simulink model "mcb_microchip_pmsm_foc_sensorless_SAME54_pot"  (R2023b)
settings: Solver=FixedStepDiscrete  StartTime=0.0  StopTime=5  FixedStep=Ts  RelTol=1e-3  EnableMultiTasking=on
InitFcn:
  | mcb_microchip_pmsm_foc_sensorless_SAME54_data
values from neighbouring files (symbols this model uses):
  PI_params = mcb.internal.SetControllerParameters(pmsm,inverter,PU_System,T_pwm,2*Ts,Ts_speed)    [mcb_microchip_pmsm_foc_sensorless_SAME54_data.m]
  PU_System = mcb_SetPUSystem(pmsm,inverter)    [mcb_microchip_pmsm_foc_sensorless_SAME54_data.m]
  PWM_frequency = 12e3    (= 12000)    [mcb_microchip_pmsm_foc_sensorless_SAME54_data.m]
  Ts = T_pwm    (= 8.33333333333e-05)    [mcb_microchip_pmsm_foc_sensorless_SAME54_data.m]
  Ts_motor = T_pwm    (= 8.33333333333e-05)    [mcb_microchip_pmsm_foc_sensorless_SAME54_data.m]
  Ts_simulink = T_pwm    (= 8.33333333333e-05)    [mcb_microchip_pmsm_foc_sensorless_SAME54_data.m]
  Ts_speed = 10*Ts    (= 0.000833333333333)    [mcb_microchip_pmsm_foc_sensorless_SAME54_data.m]
  Vd_Ref_openLoop_PU = 0.15    [mcb_microchip_pmsm_foc_sensorless_SAME54_data.m]
undefined symbols (not defined in the file or in its folder): AIN0, AIN6, DiscIntNeverNeededParam, inverter, PA02, PA03, PA06, PA08, PA09, PA10, PA11, PA12, PA13, PA16, PA17, PA18, pad0, pad1, pad2, pad3, PB08, Pin, pmsm, SAME54P20A, Timer, TQFP128, VREFA, wo0, wo1, wo2, wo4, wo5, wo6
libraries: simulink x16, MCHP_Blockset x15, mcbcontrolslib x10, slpidlib x3, mcbpositiondecoderlib x2, mcbsensorlessestimatorlib x1, mcbplantlib x1, autolibpmsmexterior x1
(part 2 of 4)

== system mcb_microchip_pmsm_foc_sensorless_SAME54_pot/Configurations ==
  note: PIM: https://www.microchip.com/Developmenttools/ProductDetails/MA320203
  note: MCLV-2				SAME70-PIM
      | --------------------------------------------------
      | DBG_LED1			PC23
      | DBG_LED2			PA24
      |
      | Rx					PA09_URXD0
      | Tx					PA10_UTXD0
      |
      | HALLA				PA00 - PD13
      | HALLB				PA01 - PD10
      | HALLC				PA16 - PD11
      |
      | PWM1				PD24 (L) - PA11 (H)
      | PWM2				PD25 (L) - PA12 (H)
      | PWM3				PD26 (L) - PA13 (H)
      |
      | FAULT				PD09_FAULT_PWM
      |
      | POT				PB00 (not ok on early PIMs)
      | PUSH S2			PC03
      | PUSH S3			PC01
      |
      | PIM_V_M1			PD30
      | PIM_V_M2			PA17
      | PIM_V_M3			PA21 - PA19
  Compiler Options : MCHP_Blockset/System Configuration/Compiler Options  Priority=1  LATEST_CMPLR=on  COMP_LIST=Dynamic Options  COMP_LIST_TXT=xc32 - v4.30  DFP_LIST=Dynamic Options  DFP_LIST_TXT=v 3.8.234  CMSIS_DSP=Dynamic Options  CMSIS_DSP_TXT=Not used  USE_64BIT_DOUBLE=off  MCHP_MULTITHREAD_COMPILATION=on  UseCustom_LinkerScript=off  MCHP_MASTERLINK=mcb_microchip_pmsm_foc_sensorless_SAME54_pot1/Configurations/Microchip Master  OPTIMIZATION_LEVEL=3  MPLAB_LINKLIB=default  MPLAB_LINKLIB1=default  CodeReplacement=Dynamic Options  CodeReplacement_TXT=None  OPTIMIZATION_FLTO=off  OPTIMIZATION_REORDER=off  UNROLL_LOOPS=on  PROCEDURAL_ABSTRACTION=off  MCODE=is less than 32768 (faster)  MCONST=in data memory  MDATA=Use only memory below address 8192 (faster)  MSCALAR=Use only memory below address 8192 (faster)  MLARGEARRAY=off  MAGGREGATE=off  HEAP_SIZE=0  OMF=elf  DEBUG_INFO=on  ProduceHexOutput=off  AssemblyListing=off  SaveTemps=off  NO_EDS_WARN=on  PRINT_STATISTICS=off
      settings: SourceProductName=MPLAB Device Blocks for Simulink
  Microchip Master : MCHP_Blockset/System Configuration/Microchip Master  Priority=1  PICREF=SAME54P20A - TQFP128  TIMESTEP_REF="Timer  ( 8.3333e-05s )"  BUSYFLAG=Dynamic Options  BUSYFLAG_TXT=None  VDD_range=Dynamic Options  PWRTEN=Not used  BOREN=Disable  BODENV=2.7V  BORV=Not used  FPWRT=64ms  DSBOREN=Enable ZPBOR during Deep Sleep Mode  DSLPBOR=Not used  MCLRE=Enabled  SMCLR=MCLR pin generates a normal system Reset  PMDL1WAY=Allow only one reconfiguration  RSTPRI=Device will obtain reset instruction from Primary flash  TEMP=Not used  SOSCSRC=Not used  SOSCSEL=Not used  IOL1WAY=Allow only one reconfiguration  ALTVREF=Not used  DISUVREG=Not used  DSSWEN=Not used  LPCFG=Not used  RTCBAT=Not used  VBTBOR=Not used  WUTSEL=Not used  POWERSAVE=off  FNOSC=Primary Oscillator with PLL module (XT + PLL; HS + PLL; EC + PLL)  FPR=ECIO w/ PLL 16x  FOSFPR=HS3 w/PLL 16x  FOS=Internal Fast RC  FRANGE=High Range  OSCILLATOR_SELECT=Crystal Oscillator in 8-48MHz on XIN/XOUT 0  OSCILLATOR_SELECT_spd=Crystal Oscillator in 8-48MHz on XIN/XOUT 0  QUARTZ=12e6  QUARTZ_spd=12e6  POSCGAIN=2x gain setting  POSCBOOST=Boost the kick start of the oscillator  SOSCGAIN=2x gain setting  SOSCBOOST=Boost the kick start of the oscillator  ACTIV_PLL=on  ACTIV_PLL_spd=on  MIPS_DESIRED=120e6  MIPS_DESIRED_spd=120e6  CPUDIV=Divide by 1  FPLLMUL=Not used  FPLLIDIV=8x Divider  POSCFREQ=Not used  POSCMD=Primary Oscillator Disabled  POSCMOD=Primary osc disabled  MIPS=120 * 1e6  ACLKCON=Optimized for PWM resolution & ADC conversion speed  ACLKCON_spd=Optimized for PWM resolution & ADC conversion speed  ACLKCON_Info=use FRC with auxilliary PLL, ADC Tad = 16.961(ns), PWM max resolution = 1.06(ns)  FPLLODIV=32x Divider  PLLKEN=Clock switch to PLL source will wait until the PLL lock signal is valid  FCKSM=Both Clock switching and Fail-safe Clock Monitor are disabled  FCKSMEN=Sw Disabled; Mon Disabled  IESO=Start up with FRC; then switch  DSWDTPS=1:2^36  FWDTEN=Disable  FWDTWINSZ=Window size is 25%  FWPSA=1:512  FWPSA0=1:128  FWPSB=1:16  WDT=Disable  WDTPOST=1:32768  WDTPRE=1:128  WDTPS=1:1048576  WINDIS=Watchdog Timer in Non-Window mode  WWDTEN=Non-Window mode  DSWDTEN=Enable DSWDT during Deep Sleep Mode  DSWDTOSC=Select LPRC as DSWDT Reference clock  FWDT_RCLKSEL=WDT Run Mode uses BFRC:256  FWDT_RWDTPS=1:2147483648  FWDT_SWDTMPS=1:2147483648  FWDT_WDTEN=WDT is controlled by software; use WDTCON.ON bit  FWDT_WDTRSTEN=WDT event generates a reset  FWDT_WDTWIN=WDT Window is 25% of WDT period  FWDT_WINEN=Watchdog Timer operates in Window mode  FPBDIV=Not used  FSOSCEN=Disable Secondary Oscillator  LPRCSEL=Not used  OSCIOFCN=Not used  OSCIOFNC=OSC2 is clock output  LVRCFG=Not used  PLL_96MHZ=Not used  PLL96MHZ=Not used  PLLDIV=Not used  WDTCLK=Not used  WDTCMX=Not used  WDTWIN=WDT Window is 25% of WDT period  XTCFG=24-32 MHz crystals  XTBST=Boost the kick-start  APL=Aux Flash Code protect is disabled  APLK=Aux Flash Write Protection or Code Protection is Enabled  AWRP=Auxiliary program memory is not write-protected  BSS=No Protection (other than BWRP)  BWP=Not used  BWRP=Boot Segment may be written  CP=Protection Disabled  EBS=No Boot EEPROM  ESS=No Segment Data EEPROM  GCP=Disable  GSS=No Protection (other than GWRP)  GSS0=Not used  GSSK=General Segment Write Protection or Code Protection is Enabled  GWRP=General Segment may be written  PWP=Not used  RBS=No Boot RAM  RSS=No Secure RAM  SSS=No Secure Segment  SWRP=Secure segment may be written  WPCFG=Not used  WPDIS=Not used  WPEND=Not used  WPFP=Not used  ICESEL=Communicate on PGEC1/PGED1  ICS=Communicate on PGEC1 and PGED1  JTAGEN=Disable  FICD_JTAGEN=Disable  COE=Not used  RES=Not used  DEBUG=Debugger is disabled  BACKBUG=Not used  BKBUG=Not used  ALTI2C=I2C mapped to SDA1/SCL1 pins  ALTI2C1=I2C1 mapped to SDA1/SCL1 pins  ALTI2C2=I2C2 mapped to SDA2/SCL2 pins  ALTI2C3=I2C3 mapped to SDA3/SCL3 pins  FDEVOPT1_ALTI2C1=Primary I2C1 pins are used  FDEVOPT1_ALTI2C2=Primary I2C2 pins are used  FDEVOPT1_SPI2MAPDIS=SPI2 pins are selected by peripheral pin selection feature  ALTQIO=QEA1; QEB1; INDX1 are selected as inputs to QEI1  ALTSS1=SS1A is selected as the I/O pin for SPI1  CMPPOL0=Hysteresis is applied to falling edge  CMPPOL1=Hysteresis is applied to falling edge  FCANIO=Not used  FETHIO=Default Ethernet I/O  FMIIEN=MII Enabled  FSRSSEL=Not used  FUSBIDIO=Controlled by the USB Module  FVBUSONIO=Not used  HPOL=Active High  HYST0=45 mV Hysteresis  HYST1=45 mV Hysteresis  I2C1SEL=Not used  LPOL=Active High  PWMPIN=Control with PORT/TRIS regs  RTCOSC=Not used  UPLLEN=USB PLL Disabled  UPLLIDIV=Not used  ATMOD8=Not used  ALTPMP=Not used  I2C2SEL=Not used  ALTADREF=Not used  ALTCVREF=Not used  PWMLOCK=PWM registers may be written without key sequence  INT_PRIORITY_DMA=0  MCHP_TIMER_RESULT=[1 8748.999999999992724 ]  MCHP_PLLRegisters="[5    243  16387     -1     -1]"  MCHPVAR=MCHP.id.name='SAME54P20A';MCHP.id.N=reshape([54 20 -1],1,3);MCHP.id.L=reshape({ 'SAME','P','A'},1,3);MCHP.id.maskset='';MCHP.id.dos='';MCHP.id.ds='';MCHP.id.archTxt='';MCHP.id.clonedfrom='';MCHP.id.Arch=6;MCHP.id.pinout=reshape({ 'TFBGA120','TQFP128'},1,2);MCHP.Rx=reshape([1 125 3 13 -1 -1 -1 -1 -1 -1 -1 -1 -1 -1 -1 -1 -1 -1 -1 -1 -1 2 126 4 16 -1 -1 -1 -1 -1 -1 -1 -1 -1 -1 -1 -1 -1 -1 -1 -1 -1 9 127 7 -1 -1 -1 -1 -1 -1 -1 -1 -1 -1 -1 -1 -1 -1 -1 -1 -1 -1 10 128 8 -1 -1 -1 -1 -1 -1 -1 -1 -1 -1 -1 -1 -1 -1 -1 -1 -1 -1 21 11 27 -1 -1 -1 -1 -1 -1 -1 -1 -1 -1 -1 -1 -1 -1 -1 -1 -1 -1 22 12 28 -1 -1 -1 -1 -1 -1 -1 -1 -1 -1 -1 -1 -1 -1 -1 -1 -1 -1 23 17 29 -1 -1 -1 -1 -1 -1 -1 -1 -1 -1 -1 -1 -1 -1 -1 -1 -1 -1 24 18 30 -1 -1 -1 -1 -1 -1 -1 -1 -1 -1 -1 -1 -1 -1 -1 -1 -1 -1 33 19 -1 47 -1 -1 -1 -1 -1 -1 -1 -1 -1 -1 -1 -1 -1 -1 -1 -1 -1 34 20 -1 48 -1 -1 -1 -1 -1 -1 -1 -1 -1 -1 -1 -1 -1 -1 -1 -1 -1 35 39 52 49 -1 -1 -1 -1 -1 -1 -1 -1 -1 -1 -1 -1 -1 -1 -1 -1 -1 36 40 55 50 -1 -1 -1 -1 -1 -1 -1 -1 -1 -1 -1 -1 -1 -1 -1 -1 -1 60 41 56 51 -1 -1 -1 -1 -1 -1 -1 -1 -1 -1 -1 -1 -1 -1 -1 -1 -1 61 42 57 -1 -1 -1 -1 -1 -1 -1 -1 -1 -1 -1 -1 -1 -1 -1 -1 -1 -1 62 43 58 -1 -1 -1 -1 -1 -1 -1 -1 -1 -1 -1 -1 -1 -1 -1 -1 -1 -1 63 44 59 -1 -1 -1 -1 -1 -1 -1 -1 -1 -1 -1 -1 -1 -1 -1 -1 -1 -1 66 82 70 -1 -1 -1 -1 -1 -1 -1 -1 -1 -1 -1 -1 -1 -1 -1 -1 -1 -1 67 83 71 -1 -1 -1 -1 -1 -1 -1 -1 -1 -1 -1 -1 -1 -1 -1 -1 -1 -1 68 84 72 -1 -1 -1 -1 -1 -1 -1 -1 -1 -1 -1 -1 -1 -1 -1 -1 -1 -1 69 85 73 -1 -1 -1 -1 -1 -1 -1 -1 -1 -1 -1 -1 -1 -1 -1 -1 -1 -1 88 86 74 80 -1 -1 -1 -1 -1 -1 -1 -1 -1 -1 -1 -1 -1 -1 -1 -1 -1 89 87 75 81 -1 -1 -1 -1 -1 -1 -1 -1 -1 -1 -1 -1 -1 -1 -1 -1 -1 92 98 76 -1 -1 -1 -1 -1 -1 -1 -1 -1 -1 -1 -1 -1 -1 -1 -1 -1 -1 93 99 77 -1 -1 -1 -1 -1 -1 -1 -1 -1 -1 -1 -1 -1 -1 -1 -1 -1 -1 94 100 108 -1 -1 -1 -1 -1 -1 -1 -1 -1 -1 -1 -1 -1 -1 -1 -1 -1 -1 95 101 109 -1 -1 -1 -1 -1 -1 -1 -1 -1 -1 -1 -1 -1 -1 -1 -1 -1 -1 -1 102 110 -1 -1 -1 -1 -1 -1 -1 -1 -1 -1 -1 -1 -1 -1 -1 -1 -1 -1 113 103 111 -1 -1 -1 -1 -1 -1 -1 -1 -1 -1 -1 -1 -1 -1 -1 -1 -1 -1 -1 104 112 -1 -1 -1 -1 -1 -1 -1 -1 -1 -1 -1 -1 -1 -1 -1 -1 -1 -1 -1 105 -1 -1 -1 -1 -1 -1 -1 -1 -1 -1 -1 -1 -1 -1 -1 -1 -1 -1 -1 119 121 123 -1 -1 -1 -1 -1 -1 -1 -1 -1 -1 -1 -1 -1 -1 -1 -1 -1 -1 120 122 124 -1 -1 -1 -1 -1 -1 -1 -1 -1 -1 -1 -1 -1 -1 -1 -1 -1 -1],21,32);MCHP.memory.FLASH.size=1048576;MCHP.memory.SW0.size=16;MCHP.memory.TEMP_LOG.size=512;MCHP.memory.USER_PAGE.size=512;MCHP.memory.CMCC.size=16777216;MCHP.memory.CMCC_DATARAM.size=4096;MCHP.memory.CMCC_TAGRAM.size=1024;MCHP.memory.CMCC_VALIDRAM.size=64;MCHP.memory.QSPI.size=16777216;MCHP.memory.HSRAM.size=262144;MCHP.memory.HSRAM_ETB.size=32768;MCHP.memory.HSRAM_RET1.size=32768;MCHP.memory.HPB0.size=17408;MCHP.memory.HPB1.size=139264;MCHP.memory.HPB2.size=15360;MCHP.memory.HPB3.size=12288;MCHP.memory.SEEPROM.size=131072;MCHP.memory.SDHC0.size=3072;MCHP.memory.SDHC1.size=3072;MCHP.memory.BKUPRAM.size=8192;MCHP.memory.PPB.size=1048576;MCHP.memory.SCS.size=4096;MCHP.memory.PERIPHERALS.size=MCHP_Fun.Hex2num('41C0000000000000');MCHP.module.PM.PID=0;MCHP.module.PM.vector='PM';MCHP.module.MCLK.PID=1;MCHP.module.MCLK.vector='MCLK';MCHP.module.OSCCTRL(1).PID=2;MCHP.module.OSCCTRL(1).vector='OSCCTRL_XOSC0';MCHP.module.OSCCTRL(1).pin.XIN0.txt={ 'PA14'};MCHP.module.OSCCTRL(1).pin.XIN0.Rx_idx=14;MCHP.module.OSCCTRL(1).pin.XIN0.ABCD=-10;MCHP.module.OSCCTRL(1).pin.XIN1.txt={ 'PB22'};MCHP.module.OSCCTRL(1).pin.XIN1.Rx_idx=54;MCHP.module.OSCCTRL(1).pin.XIN1.ABCD=-10;MCHP.module.OSCCTRL(1).pin.XOUT0.txt={ 'PA15'};MCHP.module.OSCCTRL(1).pin.XOUT0.Rx_idx=15;MCHP.module.OSCCTRL(1).pin.XOUT0.ABCD=-10;MCHP.module.OSCCTRL(1).pin.XOUT1.txt={ 'PB23'};MCHP.module.OSCCTRL(1).pin.XOUT1.Rx_idx=55;MCHP.module.OSCCTRL(1).pin.XOUT1.ABCD=-10;MCHP.module.OSCCTRL(2).PID=3;MCHP.module.OSCCTRL(2).vector='OSCCTRL_XOSC1';MCHP.module.OSCCTRL(2).pin=reshape(MCHP_Fun.Hex2num('[]'),0,0);MCHP.module.OSCCTRL(3).PID=4;MCHP.module.OSCCTRL(3).vector='OSCCTRL_DFLL';MCHP.module.OSCCTRL(3).pin=reshape(MCHP_Fun.Hex2num('[]'),0,0);MCHP.module.OSCCTRL(4).PID=5;MCHP.module.OSCCTRL(4).vector='OSCCTRL_DPLL0';MCHP.module.OSCCTRL(4).pin=reshape(MCHP_Fun.Hex2num('[]'),0,0);MCHP.module.OSCCTRL(5).PID=6;MCHP.module.OSCCTRL(5).vector='OSCCTRL_DPLL1';MCHP.module.OSCCTRL(5).pin=reshape(MCHP_Fun.Hex2num('[]'),0,0);MCHP.module.OSC32KCTRL.PID=7;MCHP.module.OSC32KCTRL.vector='OSC32KCTRL';MCHP.module.OSC32KCTRL.pin.XIN32.txt={ 'PA00'};MCHP.module.OSC32KCTRL.pin.XIN32.Rx_idx=0;MCHP.module.OSC32KCTRL.pin.XIN32.ABCD=-10;MCHP.module.OSC32KCTRL.pin.XOUT32.txt={ 'PA01'};MCHP.module.OSC32KCTRL.pin.XOUT32.Rx_idx=1;MCHP.module.OSC32KCTRL.pin.XOUT32.ABCD=-10;MCHP.module.SUPC(1).PID=8;MCHP.module.SUPC(1).vector='SUPC_OTHER';MCHP.module.SUPC(1).pin.OUT0.txt={ 'PB01'};MCHP.module.SUPC(1).pin.OUT0.Rx_idx=33;MCHP.module.SUPC(1).pin.OUT0.ABCD=-31;MCHP.module.SUPC(1).pin.OUT1.txt={ 'PB02'};MCHP.module.SUPC(1).pin.OUT1.Rx_idx=34;MCHP.module.SUPC(1).pin.OUT1.ABCD=-31;MCHP.module.SUPC(1).pin.VBAT.txt={ 'PB03'};MCHP.module.SUPC(1).pin.VBAT.Rx_idx=35;MCHP.module.SUPC(1).pin.VBAT.ABCD=-31;MCHP.module.SUPC(2).PID=9;MCHP.module.SUPC(2).vector='SUPC_BODDET';MCHP.module.SUPC(2).pin=reshape(MCHP_Fun.Hex2num('[]'),0,0);MCHP.module.WDT.PID=10;MCHP.module.WDT.vector='WDT';MCHP.module.RTC.PID=11;MCHP.module.RTC.vector='RTC';MCHP.module.RTC.pin.IN0.txt={ 'PB00'};MCHP.module.RTC.pin.IN0.Rx_idx=32;MCHP.module.RTC.pin.IN0.ABCD=-20;MCHP.module.RTC.pin.IN1.txt={ 'PB02'};MCHP.module.RTC.pin.IN1.Rx_idx=34;MCHP.module.RTC.pin.IN1.ABCD=-20;MCHP.module.RTC.pin.IN2.txt={ 'PA02'};MCHP.module.RTC.pin.IN2.Rx_idx=2;MCHP.module.RTC.pin.IN2.ABCD=-20;MCHP.module.RTC.pin.IN3.txt={ 'PC00'};MCHP.module.RTC.pin.IN3.Rx_idx=64;MCHP.module.RTC.pin.IN3.ABCD=-20;MCHP.module.RTC.pin.IN4.txt={ 'PC01'};MCHP.module.RTC.pin.IN4.Rx_idx=65;MCHP.module.RTC.pin.IN4.ABCD=-20;MCHP.module.RTC.pin.OUT.txt={ 'PB01'};MCHP.module.RTC.pin.OUT.Rx_idx=33;MCHP.module.RTC.pin.OUT.ABCD=-20;MCHP.module.EIC(1).PID=12;MCHP.module.EIC(1).vector='EIC_EXTINT_0';MCHP.module.EIC(1).pin.EXTINT0.txt=reshape({ 'PA00','PA16','PB00','PB16','PC00','PC16','PD00'},1,7);MCHP.module.EIC(1).pin.EXTINT0.Rx_idx=reshape([0 16 32 48 64 80 96],1,7);MCHP.module.EIC(1).pin.EXTINT0.ABCD=reshape([0 0 0 0 0 0 0],1,7);MCHP.module.EIC(1).pin.EXTINT1.txt=reshape({ 'PA01','PA17','PB01','PB17','PC01','PC17','PD01'},1,7);MCHP.module.EIC(1).pin.EXTINT1.Rx_idx=reshape([1 17 33 49 65 81 97],1,7);MCHP.module.EIC(1).pin.EXTINT1.ABCD=reshape([0 0 0 0 0 0 0],1,7);MCHP.module.EIC(1).pin.EXTINT2.txt=reshape({ 'PA02','PA18','PB02','PB18','PC02','PC18'},1,6);MCHP.module.EIC(1).pin.EXTINT2.Rx_idx=reshape([2 18 34 50 66 82],1,6);MCHP.module.EIC(1).pin.EXTINT2.ABCD=reshape([0 0 0 0 0 0],1,6);MCHP.module.EIC(1).pin.EXTINT3.txt=reshape({ 'PA03','PA19','PB03','PB19','PC03','PC19','PD08'},1,7);MCHP.module.EIC(1).pin.EXTINT3.Rx_idx=reshape([3 19 35 51 67 83 104],1,7);MCHP.module.EIC(1).pin.EXTINT3.ABCD=reshape([0 0 0 0 0 0 0],1,7);MCHP.module.EIC(1).pin.EXTINT4.txt=reshape({ 'PA04','PA20','PB04','PB20','PC04','PC20','PD09'},1,7);MCHP.module.EIC(1).pin.EXTINT4.Rx_idx=reshape([4 20 36 52 68 84 105],1,7);MCHP.module.EIC(1).pin.EXTINT4.ABCD=reshape([0 0 0 0 0 0 0],1,7);MCHP.module.EIC(1).pin.EXTINT5.txt=reshape({ 'PA05','PA21','PB05','PB21','PC05','PC21','PD10'},1,7);MCHP.module.EIC(1).pin.EXTINT5.Rx_idx=reshape([5 21 37 53 69 85 106],1,7);MCHP.module.EIC(1).pin.EXTINT5.ABCD=reshape([0 0 0 0 0 0 0],1,7);MCHP.module.EIC(1).pin.EXTINT6.txt=reshape({ 'PA06','PA22','PB06','PB22','PC06','PC22','PD11'},1,7);MCHP.module.EIC(1).pin.EXTINT6.Rx_idx=reshape([6 22 38 54 70 86 107],1,7);MCHP.module.EIC(1).pin.EXTINT6.ABCD=reshape([0 0 0 0 0 0 0],1,7);MCHP.module.EIC(1).pin.EXTINT7.txt=reshape({ 'PA07','PA23','PB07','PB23','PC23','PD12'},1,6);MCHP.module.EIC(1).pin.EXTINT7.Rx_idx=reshape([7 23 39 55 87 108],1,6);MCHP.module.EIC(1).pin.EXTINT7.ABCD=reshape([0 0 0 0 0 0],1,6);MCHP.module.EIC(1).pin.EXTINT8.txt=reshape({ 'PA24','PB08','PB24','PC24'},1,4);MCHP.module.EIC(1).pin.EXTINT8.Rx_idx=reshape([24 40 56 88],1,4);MCHP.module.EIC(1).pin.EXTINT8.ABCD=reshape([0 0 0 0],1,4);MCHP.module.EIC(1).pin.EXTINT9.txt=reshape({ 'PA09','PA25','PB09','PB25','PC07','PC25'},1,6);MCHP.module.EIC(1).pin.EXTINT9.Rx_idx=reshape([9 25 41 57 71 89],1,6);MCHP.module.EIC(1).pin.EXTINT9.ABCD=reshape([0 0 0 0 0 0],1,6);MCHP.module.EIC(1).pin.EXTINT10.txt=reshape({ 'PA10','PB10','PC10','PC26','PD20'},1,5);MCHP.module.EIC(1).pin.EXTINT10.Rx_idx=reshape([10 42 74 90 116],1,5);MCHP.module.EIC(1).pin.EXTINT10.ABCD=reshape([0 0 0 0 0],1,5);MCHP.module.EIC(1).pin.EXTINT11.txt=reshape({ 'PA11','PA27','PB11','PC11','PC27','PD21'},1,6);MCHP.module.EIC(1).pin.EXTINT11.Rx_idx=reshape([11 27 43 75 91 117],1,6);MCHP.module.EIC(1).pin.EXTINT11.ABCD=reshape([0 0 0 0 0 0],1,6);MCHP.module.EIC(1).pin.EXTINT12.txt=reshape({ 'PA12','PB12','PB26','PC12','PC28'},1,5);MCHP.module.EIC(1).pin.EXTINT12.Rx_idx=reshape([12 44 58 76 92],1,5);MCHP.module.EIC(1).pin.EXTINT12.ABCD=reshape([0 0 0 0 0],1,5);MCHP.module.EIC(1).pin.EXTINT13.txt=reshape({ 'PA13','PB13','PB27','PC13'},1,4);MCHP.module.EIC(1).pin.EXTINT13.Rx_idx=reshape([13 45 59 77],1,4);MCHP.module.EIC(1).pin.EXTINT13.ABCD=reshape([0 0 0 0],1,4);MCHP.module.EIC(1).pin.EXTINT14.txt=reshape({ 'PA30','PB14','PB28','PB30','PC14','PC30','PA14'},1,7);MCHP.module.EIC(1).pin.EXTINT14.Rx_idx=reshape([30 46 60 62 78 94 14],1,7);MCHP.module.EIC(1).pin.EXTINT14.ABCD=reshape([0 0 0 0 0 0 0],1,7);MCHP.module.EIC(1).pin.EXTINT15.txt=reshape({ 'PA15','PA31','PB15','PB29','PB31','PC15','PC31'},1,7);MCHP.module.EIC(1).pin.EXTINT15.Rx_idx=reshape([15 31 47 61 63 79 95],1,7);MCHP.module.EIC(1).pin.EXTINT15.ABCD=reshape([0 0 0 0 0 0 0],1,7);MCHP.module.EIC(1).pin.NMI.txt={ 'PA08'};MCHP.module.EIC(1).pin.NMI.Rx_idx=8;MCHP.module.EIC(1).pin.NMI.ABCD=0;MCHP.module.EIC(2).PID=13;MCHP.module.EIC(2).vector='EIC_EXTINT_1';MCHP.module.EIC(2).pin=reshape(MCHP_Fun.Hex2num('[]'),0,0);MCHP.module.EIC(3).PID=14;MCHP.module.EIC(3).vector='EIC_EXTINT_2';MCHP.module.EIC(3).pin=reshape(MCHP_Fun.Hex2num('[]'),0,0);MCHP.module.EIC(4).PID=15;MCHP.module.EIC(4).vector='EIC_EXTINT_3';MCHP.module.EIC(4).pin=reshape(MCHP_Fun.Hex2num('[]'),0,0);MCHP.module.EIC(5).PID=16;MCHP.module.EIC(5).vector='EIC_EXTINT_4';MCHP.module.EIC(5).pin=reshape(MCHP_Fun.Hex2num('[]'),0,0);MCHP.module.EIC(6).PID=17;MCHP.module.EIC(6).vector='EIC_EXTINT_5';MCHP.module.EIC(6).pin=reshape(MCHP_Fun.Hex2num('[]'),0,0);MCHP.module.EIC(7).PID=18;MCHP.module.EIC(7).vector='EIC_EXTINT_6';MCHP.module.EIC(7).pin=reshape(MCHP_Fun.Hex2num('[]'),0,0);MCHP.module.EIC(8).PID=19;MCHP.module.EIC(8).vector='EIC_EXTINT_7';MCHP.module.EIC(8).pin=reshape(MCHP_Fun.Hex2num('[]'),0,0);MCHP.module.EIC(9).PID=20;MCHP.module.EIC(9).vector='EIC_EXTINT_8';MCHP.module.EIC(9).pin=reshape(MCHP_Fun.Hex2num('[]'),0,0);MCHP.module.EIC(10).PID=21;MCHP.module.EIC(10).vector='EIC_EXTINT_9';MCHP.module.EIC(10).pin=reshape(MCHP_Fun.Hex2num('[]'),0,0);MCHP.module.EIC(11).PID=22;MCHP.module.EIC(11).vector='EIC_EXTINT_10';MCHP.module.EIC(11).pin=reshape(MCHP_Fun.Hex2num('[]'),0,0);MCHP.module.EIC(12).PID=23;MCHP.module.EIC(12).vector='EIC_EXTINT_11';MCHP.module.EIC(12).pin=reshape(MCHP_Fun.Hex2num('[]'),0,0);MCHP.module.EIC(13).PID=24;MCHP.module.EIC(13).vector='EIC_EXTINT_12';MCHP.module.EIC(13).pin=reshape(MCHP_Fun.Hex2num('[]'),0,0);MCHP.module.EIC(14).PID=25;MCHP.module.EIC(14).vector='EIC_EXTINT_13';MCHP.module.EIC(14).pin=reshape(MCHP_Fun.Hex2num('[]'),0,0);MCHP.module.EIC(15).PID=26;MCHP.module.EIC(15).vector='EIC_EXTINT_14';MCHP.module.EIC(15).pin=reshape(MCHP_Fun.Hex2num('[]'),0,0);MCHP.module.EIC(16).PID=27;MCHP.module.EIC(16).vector='EIC_EXTINT_15';MCHP.module.EIC(16).pin=reshape(MCHP_Fun.Hex2num('[]'),0,0);MCHP.module.FREQM.PID=28;MCHP.module.FREQM.vector='FREQM';MCHP.module.NVMCTRL(1).PID=29;MCHP.module.NVMCTRL(1).vector='NVMCTRL_0';MCHP.module.NVMCTRL(2).PID=30;MCHP.module.NVMCTRL(2).vector='NVMCTRL_1';MCHP.module.DMAC(1).PID=31;MCHP.module.DMAC(1).vector='DMAC_0';MCHP.module.DMAC(2).PID=32;MCHP.module.DMAC(2).vector='DMAC_1';MCHP.module.DMAC(3).PID=33;MCHP.module.DMAC(3).vector='DMAC_2';MCHP.module.DMAC(4).PID=34;MCHP.module.DMAC(4).vector='DMAC_3';MCHP.module.DMAC(5).PID=35;MCHP.module.DMAC(5).vector='DMAC_OTHER';MCHP.module.EVSYS(1).PID=36;MCHP.module.EVSYS(1).vector='EVSYS_0';MCHP.module.EVSYS(2).PID=37;MCHP.module.EVSYS(2).vector='EVSYS_1';MCHP.module.EVSYS(3).PID=38;MCHP.module.EVSYS(3).vector='EVSYS_2';MCHP.module.EVSYS(4).PID=39;MCHP.module.EVSYS(4).vector='EVSYS_3';MCHP.module.EVSYS(5).PID=40;MCHP.module.EVSYS(5).vector='EVSYS_OTHER';MCHP.module.PAC.PID=41;MCHP.module.PAC.vector='PAC';MCHP.module.RAMECC.PID=45;MCHP.module.RAMECC.vector='RAMECC';MCHP.module.SERCOM0(1).PID=46;MCHP.module.SERCOM0(1).vector='SERCOM0_0';MCHP.module.SERCOM0(1).pin.PAD0.txt=reshape({ 'PA04','PC17','PA08','PB24'},1,4);MCHP.module.SERCOM0(1).pin.PAD0.Rx_idx=reshape([4 81 8 56],1,4);MCHP.module.SERCOM0(1).pin.PAD0.ABCD=reshape([3 3 2 2],1,4);MCHP.module.SERCOM0(1).pin.PAD1.txt=reshape({ 'PA05','PC16','PA09','PB25'},1,4);MCHP.module.SERCOM0(1).pin.PAD1.Rx_idx=reshape([5 80 9 57],1,4);MCHP.module.SERCOM0(1).pin.PAD1.ABCD=reshape([3 3 2 2],1,4);MCHP.module.SERCOM0(1).pin.PAD2.txt=reshape({ 'PA06','PC18','PA10','PC24'},1,4);MCHP.module.SERCOM0(1).pin.PAD2.Rx_idx=reshape([6 82 10 88],1,4);MCHP.module.SERCOM0(1).pin.PAD2.ABCD=reshape([3 3 2 2],1,4);MCHP.module.SERCOM0(1).pin.PAD3.txt=reshape({ 'PA07','PC19','PA11','PC25'},1,4);MCHP.module.SERCOM0(1).pin.PAD3.Rx_idx=reshape([7 83 11 89],1,4);MCHP.module.SERCOM0(1).pin.PAD3.ABCD=reshape([3 3 2 2],1,4);MCHP.module.SERCOM0(2).PID=47;MCHP.module.SERCOM0(2).vector='SERCOM0_1';MCHP.module.SERCOM0(2).pin=reshape(MCHP_Fun.Hex2num('[]'),0,0);MCHP.module.SERCOM0(3).PID=48;MCHP.module.SERCOM0(3).vector='SERCOM0_2';MCHP.module.SERCOM0(3).pin=reshape(MCHP_Fun.Hex2num('[]'),0,0);MCHP.module.SERCOM0(4).PID=49;MCHP.module.SERCOM0(4).vector='SERCOM0_OTHER';MCHP.module.SERCOM0(4).pin=reshape(MCHP_Fun.Hex2num('[]'),0,0);MCHP.module.SERCOM1(1).PID=50;MCHP.module.SERCOM1(1).vector='SERCOM1_0';MCHP.module.SERCOM1(1).pin.PAD0.txt=reshape({ 'PA00','PA16','PC22','PC27'},1,4);MCHP.module.SERCOM1(1).pin.PAD0.Rx_idx=reshape([0 16 86 91],1,4);MCHP.module.SERCOM1(1).pin.PAD0.ABCD=reshape([3 2 2 2],1,4);MCHP.module.SERCOM1(1).pin.PAD1.txt=reshape({ 'PA01','PA17','PC23','PC28'},1,4);MCHP.module.SERCOM1(1).pin.PAD1.Rx_idx=reshape([1 17 87 92],1,4);MCHP.module.SERCOM1(1).pin.PAD1.ABCD=reshape([3 2 2 2],1,4);MCHP.module.SERCOM1(1).pin.PAD2.txt=reshape({ 'PA30','PA18','PB22','PD20'},1,4);MCHP.module.SERCOM1(1).pin.PAD2.Rx_idx=reshape([30 18 54 116],1,4);MCHP.module.SERCOM1(1).pin.PAD2.ABCD=reshape([3 2 2 2],1,4);MCHP.module.SERCOM1(1).pin.PAD3.txt=reshape({ 'PA31','PA19','PB23','PD21'},1,4);MCHP.module.SERCOM1(1).pin.PAD3.Rx_idx=reshape([31 19 55 117],1,4);MCHP.module.SERCOM1(1).pin.PAD3.ABCD=reshape([3 2 2 2],1,4);MCHP.module.SERCOM1(2).PID=51;MCHP.module.SERCOM1(2).vector='SERCOM1_1';MCHP.module.SERCOM1(2).pin=reshape(MCHP_Fun.Hex2num('[]'),0,0);MCHP.module.SERCOM1(3).PID=52;MCHP.module.SERCOM1(3).vector='SERCOM1_2';MCHP.module.SERCOM1(3).pin=reshape(MCHP_Fun.Hex2num('[]'),0,0);MCHP.module.SERCOM1(4).PID=53;MCHP.module.SERCOM1(4).vector='SERCOM1_OTHER';MCHP.module.SERCOM1(4).pin=reshape(MCHP_Fun.Hex2num('[]'),0,0);MCHP.module.SERCOM2(1).PID=54;MCHP.module.SERCOM2(1).vector='SERCOM2_0';MCHP.module.SERCOM2(1).pin.PAD0.txt=reshape({ 'PA09','PB25','PA12','PB26'},1,4);MCHP.module.SERCOM2(1).pin.PAD0.Rx_idx=reshape([9 57 12 58],1,4);MCHP.module.SERCOM2(1).pin.PAD0.ABCD=reshape([3 3 2 2],1,4);MCHP.module.SERCOM2(1).pin.PAD1.txt=reshape({ 'PA08','PB24','PA13','PB27'},1,4);MCHP.module.SERCOM2(1).pin.PAD1.Rx_idx=reshape([8 56 13 59],1,4);MCHP.module.SERCOM2(1).pin.PAD1.ABCD=reshape([3 3 2 2],1,4);MCHP.module.SERCOM2(1).pin.PAD2.txt=reshape({ 'PA10','PC24','PB28','PA14'},1,4);MCHP.module.SERCOM2(1).pin.PAD2.Rx_idx=reshape([10 88 60 14],1,4);MCHP.module.SERCOM2(1).pin.PAD2.ABCD=reshape([3 3 2 2],1,4);MCHP.module.SERCOM2(1).pin.PAD3.txt=reshape({ 'PA11','PC25','PB29','PA15'},1,4);MCHP.module.SERCOM2(1).pin.PAD3.Rx_idx=reshape([11 89 61 15],1,4);MCHP.module.SERCOM2(1).pin.PAD3.ABCD=reshape([3 3 2 2],1,4);MCHP.module.SERCOM2(2).PID=55;MCHP.module.SERCOM2(2).vector='SERCOM2_1';MCHP.module.SERCOM2(2).pin=reshape(MCHP_Fun.Hex2num('[]'),0,0);MCHP.module.SERCOM2(3).PID=56;MCHP.module.SERCOM2(3).vector='SERCOM2_2';MCHP.module.SERCOM2(3).pin=reshape(MCHP_Fun.Hex2num('[]'),0,0);MCHP.module.SERCOM2(4).PID=57;MCHP.module.SERCOM2(4).vector='SERCOM2_OTHER';MCHP.module.SERCOM2(4).pin=reshape(MCHP_Fun.Hex2num('[]'),0,0);MCHP.module.SERCOM3(1).PID=58;MCHP.module.SERCOM3(1).vector='SERCOM3_0';MCHP.module.SERCOM3(1).pin.PAD0.txt=reshape({ 'PA17','PC23','PA22','PB20'},1,4);MCHP.module.SERCOM3(1).pin.PAD0.Rx_idx=reshape([17 87 22 52],1,4);MCHP.module.SERCOM3(1).pin.PAD0.ABCD=reshape([3 3 2 2],1,4);MCHP.module.SERCOM3(1).pin.PAD1.txt=reshape({ 'PA16','PC22','PA23','PB21'},1,4);MCHP.module.SERCOM3(1).pin.PAD1.Rx_idx=reshape([16 86 23 53],1,4);MCHP.module.SERCOM3(1).pin.PAD1.ABCD=reshape([3 3 2 2],1,4);MCHP.module.SERCOM3(1).pin.PAD2.txt=reshape({ 'PA18','PA20','PD20','PA24'},1,4);MCHP.module.SERCOM3(1).pin.PAD2.Rx_idx=reshape([18 20 116 24],1,4);MCHP.module.SERCOM3(1).pin.PAD2.ABCD=reshape([3 3 3 2],1,4);MCHP.module.SERCOM3(1).pin.PAD3.txt=reshape({ 'PA19','PA21','PD21','PA25'},1,4);MCHP.module.SERCOM3(1).pin.PAD3.Rx_idx=reshape([19 21 117 25],1,4);MCHP.module.SERCOM3(1).pin.PAD3.ABCD=reshape([3 3 3 2],1,4);MCHP.module.SERCOM3(2).PID=59;MCHP.module.SERCOM3(2).vector='SERCOM3_1';MCHP.module.SERCOM3(2).pin=reshape(MCHP_Fun.Hex2num('[]'),0,0);MCHP.module.SERCOM3(3).PID=60;MCHP.module.SERCOM3(3).vector='SERCOM3_2';MCHP.module.SERCOM3(3).pin=reshape(MCHP_Fun.Hex2num('[]'),0,0);MCHP.module.SERCOM3(4).PID=61;MCHP.module.SERCOM3(4).vector='SERCOM3_OTHER';MCHP.module.SERCOM3(4).pin=reshape(MCHP_Fun.Hex2num('[]'),0,0);MCHP.module.SERCOM4(1).PID=62;MCHP.module.SERCOM4(1).vector='SERCOM4_0';MCHP.module.SERCOM4(1).pin.PAD0.txt=reshape({ 'PA13','PB08','PB27','PB12'},1,4);MCHP.module.SERCOM4(1).pin.PAD0.Rx_idx=reshape([13 40 59 44],1,4);MCHP.module.SERCOM4(1).pin.PAD0.ABCD=reshape([3 3 3 2],1,4);MCHP.module.SERCOM4(1).pin.PAD1.txt=reshape({ 'PA12','PB09','PB26','PB13'},1,4);MCHP.module.SERCOM4(1).pin.PAD1.Rx_idx=reshape([12 41 58 45],1,4);MCHP.module.SERCOM4(1).pin.PAD1.ABCD=reshape([3 3 3 2],1,4);MCHP.module.SERCOM4(1).pin.PAD2.txt=reshape({ 'PA14','PB10','PB28','PB14'},1,4);MCHP.module.SERCOM4(1).pin.PAD2.Rx_idx=reshape([14 42 60 46],1,4);MCHP.module.SERCOM4(1).pin.PAD2.ABCD=reshape([3 3 3 2],1,4);MCHP.module.SERCOM4(1).pin.PAD3.txt=reshape({ 'PB11','PB29','PA15','PB15'},1,4);MCHP.module.SERCOM4(1).pin.PAD3.Rx_idx=reshape([43 61 15 47],1,4);MCHP.module.SERCOM4(1).pin.PAD3.ABCD=reshape([3 3 3 2],1,4);MCHP.module.SERCOM4(2).PID=63;MCHP.module.SERCOM4(2).vector='SERCOM4_1';MCHP.module.SERCOM4(2).pin=reshape(MCHP_Fun.Hex2num('[]'),0,0);MCHP.module.SERCOM4(3).PID=64;MCHP.module.SERCOM4(3).vector='SERCOM4_2';MCHP.module.SERCOM4(3).pin=reshape(MCHP_Fun.Hex2num('[]'),0,0);MCHP.module.SERCOM4(4).PID=65;MCHP.module.SERCOM4(4).vector='SERCOM4_OTHER';MCHP.module.SERCOM4(4).pin=reshape(MCHP_Fun.Hex2num('[]'),0,0);MCHP.module.SERCOM5(1).PID=66;MCHP.module.SERCOM5(1).vector='SERCOM5_0';MCHP.module.SERCOM5(1).pin.PAD0.txt=reshape({ 'PA23','PB02','PB31','PB16'},1,4);MCHP.module.SERCOM5(1).pin.PAD0.Rx_idx=reshape([23 34 63 48],1,4);MCHP.module.SERCOM5(1).pin.PAD0.ABCD=reshape([3 3 3 2],1,4);MCHP.module.SERCOM5(1).pin.PAD1.txt=reshape({ 'PA22','PB03','PB30','PB17'},1,4);MCHP.module.SERCOM5(1).pin.PAD1.Rx_idx=reshape([22 35 62 49],1,4);MCHP.module.SERCOM5(1).pin.PAD1.ABCD=reshape([3 3 3 2],1,4);MCHP.module.SERCOM5(1).pin.PAD2.txt=reshape({ 'PA24','PB00','PB22','PA20','PB18'},1,5);MCHP.module.SERCOM5(1).pin.PAD2.Rx_idx=reshape([24 32 54 20 50],1,5);MCHP.module.SERCOM5(1).pin.PAD2.ABCD=reshape([3 3 3 2 2],1,5);MCHP.module.SERCOM5(1).pin.PAD3.txt=reshape({ 'PA25','PB01','PB23','PA21','PB19'},1,5);MCHP.module.SERCOM5(1).pin.PAD3.Rx_idx=reshape([25 33 55 21 51],1,5);MCHP.module.SERCOM5(1).pin.PAD3.ABCD=reshape([3 3 3 2 2],1,5);MCHP.module.SERCOM5(2).PID=67;MCHP.module.SERCOM5(2).vector='SERCOM5_1';MCHP.module.SERCOM5(2).pin=reshape(MCHP_Fun.Hex2num('[]'),0,0);MCHP.module.SERCOM5(3).PID=68;MCHP.module.SERCOM5(3).vector='SERCOM5_2';MCHP.module.SERCOM5(3).pin=reshape(MCHP_Fun.Hex2num('[]'),0,0);MCHP.module.SERCOM5(4).PID=69;MCHP.module.SERCOM5(4).vector='SERCOM5_OTHER';MCHP.module.SERCOM5(4).pin=reshape(MCHP_Fun.Hex2num('[]'),0,0);MCHP.module.SERCOM6(1).PID=70;MCHP.module.SERCOM6(1).vector='SERCOM6_0';MCHP.module.SERCOM6(1).pin.PAD0.txt=reshape({ 'PD09','PC13','PC04','PC16'},1,4);MCHP.module.SERCOM6(1).pin.PAD0.Rx_idx=reshape([105 77 68 80],1,4);MCHP.module.SERCOM6(1).pin.PAD0.ABCD=reshape([3 3 2 2],1,4);MCHP.module.SERCOM6(1).pin.PAD1.txt=reshape({ 'PD08','PC12','PC05','PC17'},1,4);MCHP.module.SERCOM6(1).pin.PAD1.Rx_idx=reshape([104 76 69 81],1,4);MCHP.module.SERCOM6(1).pin.PAD1.ABCD=reshape([3 3 2 2],1,4);MCHP.module.SERCOM6(1).pin.PAD2.txt=reshape({ 'PC14','PD10','PC06','PC10','PC18'},1,5);MCHP.module.SERCOM6(1).pin.PAD2.Rx_idx=reshape([78 106 70 74 82],1,5);MCHP.module.SERCOM6(1).pin.PAD2.ABCD=reshape([3 3 2 2 2],1,5);MCHP.module.SERCOM6(1).pin.PAD3.txt=reshape({ 'PC15','PD11','PC07','PC11','PC19'},1,5);MCHP.module.SERCOM6(1).pin.PAD3.Rx_idx=reshape([79 107 71 75 83],1,5);MCHP.module.SERCOM6(1).pin.PAD3.ABCD=reshape([3 3 2 2 2],1,5);MCHP.module.SERCOM6(2).PID=71;MCHP.module.SERCOM6(2).vector='SERCOM6_1';MCHP.module.SERCOM6(2).pin=reshape(MCHP_Fun.Hex2num('[]'),0,0);MCHP.module.SERCOM6(3).PID=72;MCHP.module.SERCOM6(3).vector='SERCOM6_2';MCHP.module.SERCOM6(3).pin=reshape(MCHP_Fun.Hex2num('[]'),0,0);MCHP.module.SERCOM6(4).PID=73;MCHP.module.SERCOM6(4).vector='SERCOM6_OTHER';MCHP.module.SERCOM6(4).pin=reshape(MCHP_Fun.Hex2num('[]'),0,0);MCHP.module.SERCOM7(1).PID=74;MCHP.module.SERCOM7(1).vector='SERCOM7_0';MCHP.module.SERCOM7(1).pin.PAD0.txt=reshape({ 'PB21','PD08','PB30','PC12'},1,4);MCHP.module.SERCOM7(1).pin.PAD0.Rx_idx=reshape([53 104 62 76],1,4);MCHP.module.SERCOM7(1).pin.PAD0.ABCD=reshape([3 2 2 2],1,4);MCHP.module.SERCOM7(1).pin.PAD1.txt=reshape({ 'PB20','PD09','PB31','PC13'},1,4);MCHP.module.SERCOM7(1).pin.PAD1.Rx_idx=reshape([52 105 63 77],1,4);MCHP.module.SERCOM7(1).pin.PAD1.ABCD=reshape([3 2 2 2],1,4);MCHP.module.SERCOM7(1).pin.PAD2.txt=reshape({ 'PB18','PC10','PC14','PD10','PA30'},1,5);MCHP.module.SERCOM7(1).pin.PAD2.Rx_idx=reshape([50 74 78 106 30],1,5);MCHP.module.SERCOM7(1).pin.PAD2.ABCD=reshape([3 3 2 2 2],1,5);MCHP.module.SERCOM7(1).pin.PAD3.txt=reshape({ 'PB19','PC11','PC15','PD11','PA31'},1,5);MCHP.module.SERCOM7(1).pin.PAD3.Rx_idx=reshape([51 75 79 107 31],1,5);MCHP.module.SERCOM7(1).pin.PAD3.ABCD=reshape([3 3 2 2 2],1,5);MCHP.module.SERCOM7(2).PID=75;MCHP.module.SERCOM7(2).vector='SERCOM7_1';MCHP.module.SERCOM7(2).pin=reshape(MCHP_Fun.Hex2num('[]'),0,0);MCHP.module.SERCOM7(3).PID=76;MCHP.module.SERCOM7(3).vector='SERCOM7_2';MCHP.module.SERCOM7(3).pin=reshape(MCHP_Fun.Hex2num('[]'),0,0);MCHP.module.SERCOM7(4).PID=77;MCHP.module.SERCOM7(4).vector='SERCOM7_OTHER';MCHP.module.SERCOM7(4).pin=reshape(MCHP_Fun.Hex2num('[]'),0,0);MCHP.module.CAN0.PID=78;MCHP.module.CAN0.vector='CAN0';MCHP.module.CAN0.pin.RX.txt=reshape({ 'PA23','PA25'},1,2);MCHP.module.CAN0.pin.RX.Rx_idx=reshape([23 25],1,2);MCHP.module.CAN0.pin.RX.ABCD=reshape([8 8],1,2);MCHP.module.CAN0.pin.TX.txt=reshape({ 'PA22','PA24'},1,2);MCHP.module.CAN0.pin.TX.Rx_idx=reshape([22 24],1,2);MCHP.module.CAN0.pin.TX.ABCD=reshape([8 8],1,2);MCHP.module.CAN1.PID=79;MCHP.module.CAN1.vector='CAN1';MCHP.module.CAN1.pin.RX.txt=reshape({ 'PB13','PB15'},1,2);MCHP.module.CAN1.pin.RX.Rx_idx=reshape([45 47],1,2);MCHP.module.CAN1.pin.RX.ABCD=reshape([7 7],1,2);MCHP.module.CAN1.pin.TX.txt=reshape({ 'PB12','PB14'},1,2);MCHP.module.CAN1.pin.TX.Rx_idx=reshape([44 46],1,2);MCHP.module.CAN1.pin.TX.ABCD=reshape([7 7],1,2);MCHP.module.USB(1).PID=80;MCHP.module.USB(1).vector='USB_OTHER';MCHP.module.USB(1).pin.DM.txt={ 'PA24'};MCHP.module.USB(1).pin.DM.Rx_idx=24;MCHP.module.USB(1).pin.DM.ABCD=7;MCHP.module.USB(1).pin.DP.txt={ 'PA25'};MCHP.module.USB(1).pin.DP.Rx_idx=25;MCHP.module.USB(1).pin.DP.ABCD=7;MCHP.module.USB(1).pin.SOF_1KHZ.txt=reshape({ 'PA23','PB22'},1,2);MCHP.module.USB(1).pin.SOF_1KHZ.Rx_idx=reshape([23 54],1,2);MCHP.module.USB(1).pin.SOF_1KHZ.ABCD=reshape([7 7],1,2);MCHP.module.USB(2).PID=81;MCHP.module.USB(2).vector='USB_SOF_HSOF';MCHP.module.USB(2).pin=reshape(MCHP_Fun.Hex2num('[]'),0,0);MCHP.module.USB(3).PID=82;MCHP.module.USB(3).vector='USB_TRCPT0';MCHP.module.USB(3).pin=reshape(MCHP_Fun.Hex2num('[]'),0,0);MCHP.module.USB(4).PID=83;MCHP.module.USB(4).vector='USB_TRCPT1';MCHP.module.USB(4).pin=reshape(MCHP_Fun.Hex2num('[]'),0,0);MCHP.module.GMAC.PID=84;MCHP.module.GMAC.vector='GMAC';MCHP.module.GMAC.pin.GCOL.txt={ 'PC21'};MCHP.module.GMAC.pin.GCOL.Rx_idx=85;MCHP.module.GMAC.pin.GCOL.ABCD=11;MCHP.module.GMAC.pin.GCRS.txt={ 'PA16'};MCHP.module.GMAC.pin.GCRS.Rx_idx=16;MCHP.module.GMAC.pin.GCRS.ABCD=11;MCHP.module.GMAC.pin.GMDC.txt=reshape({ 'PA20','PB14','PC11','PC22'},1,4);MCHP.module.GMAC.pin.GMDC.Rx_idx=reshape([20 46 75 86],1,4);MCHP.module.GMAC.pin.GMDC.ABCD=reshape([11 11 11 11],1,4);MCHP.module.GMAC.pin.GMDIO.txt=reshape({ 'PA21','PB15','PC12','PC23'},1,4);MCHP.module.GMAC.pin.GMDIO.Rx_idx=reshape([21 47 76 87],1,4);MCHP.module.GMAC.pin.GMDIO.ABCD=reshape([11 11 11 11],1,4);MCHP.module.GMAC.pin.GRX0.txt={ 'PA13'};MCHP.module.GMAC.pin.GRX0.Rx_idx=13;MCHP.module.GMAC.pin.GRX0.ABCD=11;MCHP.module.GMAC.pin.GRX1.txt={ 'PA12'};MCHP.module.GMAC.pin.GRX1.Rx_idx=12;MCHP.module.GMAC.pin.GRX1.ABCD=11;MCHP.module.GMAC.pin.GRX2.txt={ 'PC15'};MCHP.module.GMAC.pin.GRX2.Rx_idx=79;MCHP.module.GMAC.pin.GRX2.ABCD=11;MCHP.module.GMAC.pin.GRX3.txt={ 'PC14'};MCHP.module.GMAC.pin.GRX3.Rx_idx=78;MCHP.module.GMAC.pin.GRX3.ABCD=11;MCHP.module.GMAC.pin.GRXCK.txt={ 'PC18'};MCHP.module.GMAC.pin.GRXCK.Rx_idx=82;MCHP.module.GMAC.pin.GRXCK.ABCD=11;MCHP.module.GMAC.pin.GRXDV.txt={ 'PC20'};MCHP.module.GMAC.pin.GRXDV.Rx_idx=84;MCHP.module.GMAC.pin.GRXDV.ABCD=11;MCHP.module.GMAC.pin.GRXER.txt={ 'PA15'};MCHP.module.GMAC.pin.GRXER.Rx_idx=15;MCHP.module.GMAC.pin.GRXER.ABCD=11;MCHP.module.GMAC.pin.GTX0.txt={ 'PA18'};MCHP.module.GMAC.pin.GTX0.Rx_idx=18;MCHP.module.GMAC.pin.GTX0.ABCD=11;MCHP.module.GMAC.pin.GTX1.txt={ 'PA19'};MCHP.module.GMAC.pin.GTX1.Rx_idx=19;MCHP.module.GMAC.pin.GTX1.ABCD=11;MCHP.module.GMAC.pin.GTX2.txt={ 'PC16'};MCHP.module.GMAC.pin.GTX2.Rx_idx=80;MCHP.module.GMAC.pin.GTX2.ABCD=11;MCHP.module.GMAC.pin.GTX3.txt={ 'PC17'};MCHP.module.GMAC.pin.GTX3.Rx_idx=81;MCHP.module.GMAC.pin.GTX3.ABCD=11;MCHP.module.GMAC.pin.GTXCK.txt={ 'PA14'};MCHP.module.GMAC.pin.GTXCK.Rx_idx=14;MCHP.module.GMAC.pin.GTXCK.ABCD=11;MCHP.module.GMAC.pin.GTXEN.txt={ 'PA17'};MCHP.module.GMAC.pin.GTXEN.Rx_idx=17;MCHP.module.GMAC.pin.GTXEN.ABCD=11;MCHP.module.GMAC.pin.GTXER.txt={ 'PC19'};MCHP.module.GMAC.pin.GTXER.Rx_idx=83;MCHP.module.GMAC.pin.GTXER.ABCD=11;MCHP.module.TCC0(1).PID=85;MCHP.module.TCC0(1).vector='TCC0_OTHER';MCHP.module.TCC0(1).pin.WO0.txt=reshape({ 'PA20','PB12','PA08','PC04','PC10','PC16'},1,6);MCHP.module.TCC0(1).pin.WO0.Rx_idx=reshape([20 44 8 68 74 80],1,6);MCHP.module.TCC0(1).pin.WO0.ABCD=reshape([6 6 5 5 5 5],1,6);MCHP.module.TCC0(1).pin.WO1.txt=reshape({ 'PA21','PB13','PA09','PC11','PC17','PD08'},1,6);MCHP.module.TCC0(1).pin.WO1.Rx_idx=reshape([21 45 9 75 81 104],1,6);MCHP.module.TCC0(1).pin.WO1.ABCD=reshape([6 6 5 5 5 5],1,6);MCHP.module.TCC0(1).pin.WO2.txt=reshape({ 'PA22','PB14','PA10','PC12','PC18','PD09'},1,6);MCHP.module.TCC0(1).pin.WO2.Rx_idx=reshape([22 46 10 76 82 105],1,6);MCHP.module.TCC0(1).pin.WO2.ABCD=reshape([6 6 5 5 5 5],1,6);MCHP.module.TCC0(1).pin.WO3.txt=reshape({ 'PA23','PB15','PA11','PC13','PC19','PD10'},1,6);MCHP.module.TCC0(1).pin.WO3.Rx_idx=reshape([23 47 11 77 83 106],1,6);MCHP.module.TCC0(1).pin.WO3.ABCD=reshape([6 6 5 5 5 5],1,6);MCHP.module.TCC0(1).pin.WO4.txt=reshape({ 'PA16','PB16','PB10','PC14','PC20','PD11'},1,6);MCHP.module.TCC0(1).pin.WO4.Rx_idx=reshape([16 48 42 78 84 107],1,6);MCHP.module.TCC0(1).pin.WO4.ABCD=reshape([6 6 5 5 5 5],1,6);MCHP.module.TCC0(1).pin.WO5.txt=reshape({ 'PA17','PB17','PB11','PC15','PC21','PD12'},1,6);MCHP.module.TCC0(1).pin.WO5.Rx_idx=reshape([17 49 43 79 85 108],1,6);MCHP.module.TCC0(1).pin.WO5.ABCD=reshape([6 6 5 5 5 5],1,6);MCHP.module.TCC0(1).pin.WO6.txt=reshape({ 'PA18','PB30','PA12','PC22'},1,4);MCHP.module.TCC0(1).pin.WO6.Rx_idx=reshape([18 62 12 86],1,4);MCHP.module.TCC0(1).pin.WO6.ABCD=reshape([6 6 5 5],1,4);MCHP.module.TCC0(1).pin.WO7.txt=reshape({ 'PA19','PB31','PA13','PC23'},1,4);MCHP.module.TCC0(1).pin.WO7.Rx_idx=reshape([19 63 13 87],1,4);MCHP.module.TCC0(1).pin.WO7.ABCD=reshape([6 6 5 5],1,4);MCHP.module.TCC0(2).PID=86;MCHP.module.TCC0(2).vector='TCC0_MC0';MCHP.module.TCC0(2).pin=reshape(MCHP_Fun.Hex2num('[]'),0,0);MCHP.module.TCC0(3).PID=87;MCHP.module.TCC0(3).vector='TCC0_MC1';MCHP.module.TCC0(3).pin=reshape(MCHP_Fun.Hex2num('[]'),0,0);MCHP.module.TCC0(4).PID=88;MCHP.module.TCC0(4).vector='TCC0_MC2';MCHP.module.TCC0(4).pin=reshape(MCHP_Fun.Hex2num('[]'),0,0);MCHP.module.TCC0(5).PID=89;MCHP.module.TCC0(5).vector='TCC0_MC3';MCHP.module.TCC0(5).pin=reshape(MCHP_Fun.Hex2num('[]'),0,0);MCHP.module.TCC0(6).PID=90;MCHP.module.TCC0(6).vector='TCC0_MC4';MCHP.module.TCC0(6).pin=reshape(MCHP_Fun.Hex2num('[]'),0,0);MCHP.module.TCC0(7).PID=91;MCHP.module.TCC0(7).vector='TCC0_MC5';MCHP.module.TCC0(7).pin=reshape(MCHP_Fun.Hex2num('[]'),0,0);MCHP.module.TCC1(1).PID=92;MCHP.module.TCC1(1).vector='TCC1_OTHER';MCHP.module.TCC1(1).pin.WO0.txt=reshape({ 'PB10','PC14','PA16','PB18','PD20'},1,5);MCHP.module.TCC1(1).pin.WO0.Rx_idx=reshape([42 78 16 50 116],1,5);MCHP.module.TCC1(1).pin.WO0.ABCD=reshape([6 6 5 5 5],1,5);MCHP.module.TCC1(1).pin.WO1.txt=reshape({ 'PB11','PC15','PA17','PB19','PD21'},1,5);MCHP.module.TCC1(1).pin.WO1.Rx_idx=reshape([43 79 17 51 117],1,5);MCHP.module.TCC1(1).pin.WO1.ABCD=reshape([6 6 5 5 5],1,5);MCHP.module.TCC1(1).pin.WO2.txt=reshape({ 'PA12','PA14','PA18','PB20','PB26'},1,5);MCHP.module.TCC1(1).pin.WO2.Rx_idx=reshape([12 14 18 52 58],1,5);MCHP.module.TCC1(1).pin.WO2.ABCD=reshape([6 6 5 5 5],1,5);MCHP.module.TCC1(1).pin.WO3.txt=reshape({ 'PA13','PA15','PA19','PB21','PB27'},1,5);MCHP.module.TCC1(1).pin.WO3.Rx_idx=reshape([13 15 19 53 59],1,5);MCHP.module.TCC1(1).pin.WO3.ABCD=reshape([6 6 5 5 5],1,5);MCHP.module.TCC1(1).pin.WO4.txt=reshape({ 'PA08','PC10','PA20','PB28'},1,4);MCHP.module.TCC1(1).pin.WO4.Rx_idx=reshape([8 74 20 60],1,4);MCHP.module.TCC1(1).pin.WO4.ABCD=reshape([6 6 5 5],1,4);MCHP.module.TCC1(1).pin.WO5.txt=reshape({ 'PA09','PC11','PA21','PB29'},1,4);MCHP.module.TCC1(1).pin.WO5.Rx_idx=reshape([9 75 21 61],1,4);MCHP.module.TCC1(1).pin.WO5.ABCD=reshape([6 6 5 5],1,4);MCHP.module.TCC1(1).pin.WO6.txt=reshape({ 'PA10','PC12','PA22'},1,3);MCHP.module.TCC1(1).pin.WO6.Rx_idx=reshape([10 76 22],1,3);MCHP.module.TCC1(1).pin.WO6.ABCD=reshape([6 6 5],1,3);MCHP.module.TCC1(1).pin.WO7.txt=reshape({ 'PA11','PC13','PA23'},1,3);MCHP.module.TCC1(1).pin.WO7.Rx_idx=reshape([11 77 23],1,3);MCHP.module.TCC1(1).pin.WO7.ABCD=reshape([6 6 5],1,3);MCHP.module.TCC1(2).PID=93;MCHP.module.TCC1(2).vector='TCC1_MC0';MCHP.module.TCC1(2).pin=reshape(MCHP_Fun.Hex2num('[]'),0,0);MCHP.module.TCC1(3).PID=94;MCHP.module.TCC1(3).vector='TCC1_MC1';MCHP.module.TCC1(3).pin=reshape(MCHP_Fun.Hex2num('[]'),0,0);MCHP.module.TCC1(4).PID=95;MCHP.module.TCC1(4).vector='TCC1_MC2';MCHP.module.TCC1(4).pin=reshape(MCHP_Fun.Hex2num('[]'),0,0);MCHP.module.TCC1(5).PID=96;MCHP.module.TCC1(5).vector='TCC1_MC3';MCHP.module.TCC1(5).pin=reshape(MCHP_Fun.Hex2num('[]'),0,0);MCHP.module.TCC2(1).PID=97;MCHP.module.TCC2(1).vector='TCC2_OTHER';MCHP.module.TCC2(1).pin.WO0.txt=reshape({ 'PA14','PA30'},1,2);MCHP.module.TCC2(1).pin.WO0.Rx_idx=reshape([14 30],1,2);MCHP.module.TCC2(1).pin.WO0.ABCD=reshape([5 5],1,2);MCHP.module.TCC2(1).pin.WO1.txt=reshape({ 'PA15','PA31'},1,2);MCHP.module.TCC2(1).pin.WO1.Rx_idx=reshape([15 31],1,2);MCHP.module.TCC2(1).pin.WO1.ABCD=reshape([5 5],1,2);MCHP.module.TCC2(1).pin.WO2.txt=reshape({ 'PA24','PB02'},1,2);MCHP.module.TCC2(1).pin.WO2.Rx_idx=reshape([24 34],1,2);MCHP.module.TCC2(1).pin.WO2.ABCD=reshape([5 5],1,2);MCHP.module.TCC2(2).PID=98;MCHP.module.TCC2(2).vector='TCC2_MC0';MCHP.module.TCC2(2).pin=reshape(MCHP_Fun.Hex2num('[]'),0,0);MCHP.module.TCC2(3).PID=99;MCHP.module.TCC2(3).vector='TCC2_MC1';MCHP.module.TCC2(3).pin=reshape(MCHP_Fun.Hex2num('[]'),0,0);MCHP.module.TCC2(4).PID=100;MCHP.module.TCC2(4).vector='TCC2_MC2';MCHP.module.TCC2(4).pin=reshape(MCHP_Fun.Hex2num('[]'),0,0);MCHP.module.TCC3(1).PID=101;MCHP.module.TCC3(1).vector='TCC3_OTHER';MCHP.module.TCC3(1).pin.WO0.txt=reshape({ 'PB12','PB16'},1,2);MCHP.module.TCC3(1).pin.WO0.Rx_idx=reshape([44 48],1,2);MCHP.module.TCC3(1).pin.WO0.ABCD=reshape([5 5],1,2);MCHP.module.TCC3(1).pin.WO1.txt=reshape({ 'PB13','PB17'},1,2);MCHP.module.TCC3(1).pin.WO1.Rx_idx=reshape([45 49],1,2);MCHP.module.TCC3(1).pin.WO1.ABCD=reshape([5 5],1,2);MCHP.module.TCC3(2).PID=102;MCHP.module.TCC3(2).vector='TCC3_MC0';MCHP.module.TCC3(2).pin=reshape(MCHP_Fun.Hex2num('[]'),0,0);MCHP.module.TCC3(3).PID=103;MCHP.module.TCC3(3).vector='TCC3_MC1';MCHP.module.TCC3(3).pin=reshape(MCHP_Fun.Hex2num('[]'),0,0);MCHP.module.TCC4(1).PID=104;MCHP.module.TCC4(1).vector='TCC4_OTHER';MCHP.module.TCC4(1).pin.WO0.txt=reshape({ 'PB14','PB30'},1,2);MCHP.module.TCC4(1).pin.WO0.Rx_idx=reshape([46 62],1,2);MCHP.module.TCC4(1).pin.WO0.ABCD=reshape([5 5],1,2);MCHP.module.TCC4(1).pin.WO1.txt=reshape({ 'PB15','PB31'},1,2);MCHP.module.TCC4(1).pin.WO1.Rx_idx=reshape([47 63],1,2);MCHP.module.TCC4(1).pin.WO1.ABCD=reshape([5 5],1,2);MCHP.module.TCC4(2).PID=105;MCHP.module.TCC4(2).vector='TCC4_MC0';MCHP.module.TCC4(2).pin=reshape(MCHP_Fun.Hex2num('[]'),0,0);MCHP.module.TCC4(3).PID=106;MCHP.module.TCC4(3).vector='TCC4_MC1';MCHP.module.TCC4(3).pin=reshape(MCHP_Fun.Hex2num('[]'),0,0);MCHP.module.TC0.PID=107;MCHP.module.TC0.vector='TC0';MCHP.module.TC0.pin.WO0.txt=reshape({ 'PA04','PA08','PB30'},1,3);MCHP.module.TC0.pin.WO0.Rx_idx=reshape([4 8 62],1,3);MCHP.module.TC0.pin.WO0.ABCD=reshape([4 4 4],1,3);MCHP.module.TC0.pin.WO1.txt=reshape({ 'PA05','PA09','PB31'},1,3);MCHP.module.TC0.pin.WO1.Rx_idx=reshape([5 9 63],1,3);MCHP.module.TC0.pin.WO1.ABCD=reshape([4 4 4],1,3);MCHP.module.TC1.PID=108;MCHP.module.TC1.vector='TC1';MCHP.module.TC1.pin.WO0.txt=reshape({ 'PA06','PA10'},1,2);MCHP.module.TC1.pin.WO0.Rx_idx=reshape([6 10],1,2);MCHP.module.TC1.pin.WO0.ABCD=reshape([4 4],1,2);MCHP.module.TC1.pin.WO1.txt=reshape({ 'PA07','PA11'},1,2);MCHP.module.TC1.pin.WO1.Rx_idx=reshape([7 11],1,2);MCHP.module.TC1.pin.WO1.ABCD=reshape([4 4],1,2);MCHP.module.TC2.PID=109;MCHP.module.TC2.vector='TC2';MCHP.module.TC2.pin.WO0.txt=reshape({ 'PA12','PA16','PA00'},1,3);MCHP.module.TC2.pin.WO0.Rx_idx=reshape([12 16 0],1,3);MCHP.module.TC2.pin.WO0.ABCD=reshape([4 4 4],1,3);MCHP.module.TC2.pin.WO1.txt=reshape({ 'PA01','PA13','PA17'},1,3);MCHP.module.TC2.pin.WO1.Rx_idx=reshape([1 13 17],1,3);MCHP.module.TC2.pin.WO1.ABCD=reshape([4 4 4],1,3);MCHP.module.TC3.PID=110;MCHP.module.TC3.vector='TC3';MCHP.module.TC3.pin.WO0.txt=reshape({ 'PA18','PA14'},1,2);MCHP.module.TC3.pin.WO0.Rx_idx=reshape([18 14],1,2);MCHP.module.TC3.pin.WO0.ABCD=reshape([4 4],1,2);MCHP.module.TC3.pin.WO1.txt=reshape({ 'PA15','PA19'},1,2);MCHP.module.TC3.pin.WO1.Rx_idx=reshape([15 19],1,2);MCHP.module.TC3.pin.WO1.ABCD=reshape([4 4],1,2);MCHP.module.TC4.PID=111;MCHP.module.TC4.vector='TC4';MCHP.module.TC4.pin.WO0.txt=reshape({ 'PA22','PB08','PB12'},1,3);MCHP.module.TC4.pin.WO0.Rx_idx=reshape([22 40 44],1,3);MCHP.module.TC4.pin.WO0.ABCD=reshape([4 4 4],1,3);MCHP.module.TC4.pin.WO1.txt=reshape({ 'PA23','PB09','PB13'},1,3);MCHP.module.TC4.pin.WO1.Rx_idx=reshape([23 41 45],1,3);MCHP.module.TC4.pin.WO1.ABCD=reshape([4 4 4],1,3);MCHP.module.TC5.PID=112;MCHP.module.TC5.vector='TC5';MCHP.module.TC5.pin.WO0.txt=reshape({ 'PA24','PB10','PB14'},1,3);MCHP.module.TC5.pin.WO0.Rx_idx=reshape([24 42 46],1,3);MCHP.module.TC5.pin.WO0.ABCD=reshape([4 4 4],1,3);MCHP.module.TC5.pin.WO1.txt=reshape({ 'PA25','PB11','PB15'},1,3);MCHP.module.TC5.pin.WO1.Rx_idx=reshape([25 43 47],1,3);MCHP.module.TC5.pin.WO1.ABCD=reshape([4 4 4],1,3);MCHP.module.TC6.PID=113;MCHP.module.TC6.vector='TC6';MCHP.module.TC6.pin.WO0.txt=reshape({ 'PA30','PB02','PB16'},1,3);MCHP.module.TC6.pin.WO0.Rx_idx=reshape([30 34 48],1,3);MCHP.module.TC6.pin.WO0.ABCD=reshape([4 4 4],1,3);MCHP.module.TC6.pin.WO1.txt=reshape({ 'PA31','PB03','PB17'},1,3);MCHP.module.TC6.pin.WO1.Rx_idx=reshape([31 35 49],1,3);MCHP.module.TC6.pin.WO1.ABCD=reshape([4 4 4],1,3);MCHP.module.TC7.PID=114;MCHP.module.TC7.vector='TC7';MCHP.module.TC7.pin.WO0.txt=reshape({ 'PA20','PB00','PB22'},1,3);MCHP.module.TC7.pin.WO0.Rx_idx=reshape([20 32 54],1,3);MCHP.module.TC7.pin.WO0.ABCD=reshape([4 4 4],1,3);MCHP.module.TC7.pin.WO1.txt=reshape({ 'PA21','PB01','PB23'},1,3);MCHP.module.TC7.pin.WO1.Rx_idx=reshape([21 33 55],1,3);MCHP.module.TC7.pin.WO1.ABCD=reshape([4 4 4],1,3);MCHP.module.PDEC(1).PID=115;MCHP.module.PDEC(1).vector='PDEC_OTHER';MCHP.module.PDEC(1).pin.QDI0.txt=reshape({ 'PB18','PB23','PC16','PA24'},1,4);MCHP.module.PDEC(1).pin.QDI0.Rx_idx=reshape([50 55 80 24],1,4);MCHP.module.PDEC(1).pin.QDI0.ABCD=reshape([6 6 6 6],1,4);MCHP.module.PDEC(1).pin.QDI1.txt=reshape({ 'PB19','PB24','PC17','PA25'},1,4);MCHP.module.PDEC(1).pin.QDI1.Rx_idx=reshape([51 56 81 25],1,4);MCHP.module.PDEC(1).pin.QDI1.ABCD=reshape([6 6 6 6],1,4);MCHP.module.PDEC(1).pin.QDI2.txt=reshape({ 'PB20','PB25','PC18','PB22'},1,4);MCHP.module.PDEC(1).pin.QDI2.Rx_idx=reshape([52 57 82 54],1,4);MCHP.module.PDEC(1).pin.QDI2.ABCD=reshape([6 6 6 6],1,4);MCHP.module.PDEC(2).PID=116;MCHP.module.PDEC(2).vector='PDEC_MC0';MCHP.module.PDEC(2).pin=reshape(MCHP_Fun.Hex2num('[]'),0,0);MCHP.module.PDEC(3).PID=117;MCHP.module.PDEC(3).vector='PDEC_MC1';MCHP.module.PDEC(3).pin=reshape(MCHP_Fun.Hex2num('[]'),0,0);MCHP.module.ADC0(1).PID=118;MCHP.module.ADC0(1).vector='ADC0_OTHER';MCHP.module.ADC0(1).pin.AIN0.txt={ 'PA02'};MCHP.module.ADC0(1).pin.AIN0.Rx_idx=2;MCHP.module.ADC0(1).pin.AIN0.ABCD=1;MCHP.module.ADC0(1).pin.AIN1.txt={ 'PA03'};MCHP.module.ADC0(1).pin.AIN1.Rx_idx=3;MCHP.module.ADC0(1).pin.AIN1.ABCD=1;MCHP.module.ADC0(1).pin.AIN2.txt={ 'PB08'};MCHP.module.ADC0(1).pin.AIN2.Rx_idx=40;MCHP.module.ADC0(1).pin.AIN2.ABCD=1;MCHP.module.ADC0(1).pin.AIN3.txt={ 'PB09'};MCHP.module.ADC0(1).pin.AIN3.Rx_idx=41;MCHP.module.ADC0(1).pin.AIN3.ABCD=1;MCHP.module.ADC0(1).pin.AIN4.txt={ 'PA04'};MCHP.module.ADC0(1).pin.AIN4.Rx_idx=4;MCHP.module.ADC0(1).pin.AIN4.ABCD=1;MCHP.module.ADC0(1).pin.AIN5.txt={ 'PA05'};MCHP.module.ADC0(1).pin.AIN5.Rx_idx=5;MCHP.module.ADC0(1).pin.AIN5.ABCD=1;MCHP.module.ADC0(1).pin.AIN6.txt={ 'PA06'};MCHP.module.ADC0(1).pin.AIN6.Rx_idx=6;MCHP.module.ADC0(1).pin.AIN6.ABCD=1;MCHP.module.ADC0(1).pin.AIN7.txt={ 'PA07'};MCHP.module.ADC0(1).pin.AIN7.Rx_idx=7;MCHP.module.ADC0(1).pin.AIN7.ABCD=1;MCHP.module.ADC0(1).pin.AIN8.txt={ 'PA08'};MCHP.module.ADC0(1).pin.AIN8.Rx_idx=8;MCHP.module.ADC0(1).pin.AIN8.ABCD=1;MCHP.module.ADC0(1).pin.AIN9.txt={ 'PA09'};MCHP.module.ADC0(1).pin.AIN9.Rx_idx=9;MCHP.module.ADC0(1).pin.AIN9.ABCD=1;MCHP.module.ADC0(1).pin.AIN10.txt={ 'PA10'};MCHP.module.ADC0(1).pin.AIN10.Rx_idx=10;MCHP.module.ADC0(1).pin.AIN10.ABCD=1;MCHP.module.ADC0(1).pin.AIN11.txt={ 'PA11'};MCHP.module.ADC0(1).pin.AIN11.Rx_idx=11;MCHP.module.ADC0(1).pin.AIN11.ABCD=1;MCHP.module.ADC0(1).pin.AIN12.txt={ 'PB00'};MCHP.module.ADC0(1).pin.AIN12.Rx_idx=32;MCHP.module.ADC0(1).pin.AIN12.ABCD=1;MCHP.module.ADC0(1).pin.AIN13.txt={ 'PB01'};MCHP.module.ADC0(1).pin.AIN13.Rx_idx=33;MCHP.module.ADC0(1).pin.AIN13.ABCD=1;MCHP.module.ADC0(1).pin.AIN14.txt={ 'PB02'};MCHP.module.ADC0(1).pin.AIN14.Rx_idx=34;MCHP.module.ADC0(1).pin.AIN14.ABCD=1;MCHP.module.ADC0(1).pin.AIN15.txt={ 'PB03'};MCHP.module.ADC0(1).pin.AIN15.Rx_idx=35;MCHP.module.ADC0(1).pin.AIN15.ABCD=1;MCHP.module.ADC0(1).pin.X0.txt={ 'PA03'};MCHP.module.ADC0(1).pin.X0.Rx_idx=3;MCHP.module.ADC0(1).pin.X0.ABCD=1;MCHP.module.ADC0(1).pin.Y0.txt={ 'PA03'};MCHP.module.ADC0(1).pin.Y0.Rx_idx=3;MCHP.module.ADC0(1).pin.Y0.ABCD=1;MCHP.module.ADC0(1).pin.X1.txt={ 'PB08'};MCHP.module.ADC0(1).pin.X1.Rx_idx=40;MCHP.module.ADC0(1).pin.X1.ABCD=1;MCHP.module.ADC0(1).pin.Y1.txt={ 'PB08'};MCHP.module.ADC0(1).pin.Y1.Rx_idx=40;MCHP.module.ADC0(1).pin.Y1.ABCD=1;MCHP.module.ADC0(1).pin.X2.txt={ 'PB09'};MCHP.module.ADC0(1).pin.X2.Rx_idx=41;MCHP.module.ADC0(1).pin.X2.ABCD=1;MCHP.module.ADC0(1).pin.Y2.txt={ 'PB09'};MCHP.module.ADC0(1).pin.Y2.Rx_idx=41;MCHP.module.ADC0(1).pin.Y2.ABCD=1;MCHP.module.ADC0(1).pin.X3.txt={ 'PA04'};MCHP.module.ADC0(1).pin.X3.Rx_idx=4;MCHP.module.ADC0(1).pin.X3.ABCD=1;MCHP.module.ADC0(1).pin.Y3.txt={ 'PA04'};MCHP.module.ADC0(1).pin.Y3.Rx_idx=4;MCHP.module.ADC0(1).pin.Y3.ABCD=1;MCHP.module.ADC0(1).pin.X4.txt={ 'PA06'};MCHP.module.ADC0(1).pin.X4.Rx_idx=6;MCHP.module.ADC0(1).pin.X4.ABCD=1;MCHP.module.ADC0(1).pin.Y4.txt={ 'PA06'};MCHP.module.ADC0(1).pin.Y4.Rx_idx=6;MCHP.module.ADC0(1).pin.Y4.ABCD=1;MCHP.module.ADC0(1).pin.X5.txt={ 'PA07'};MCHP.module.ADC0(1).pin.X5.Rx_idx=7;MCHP.module.ADC0(1).pin.X5.ABCD=1;MCHP.module.ADC0(1).pin.Y5.txt={ 'PA07'};MCHP.module.ADC0(1).pin.Y5.Rx_idx=7;MCHP.module.ADC0(1).pin.Y5.ABCD=1;MCHP.module.ADC0(1).pin.X6.txt={ 'PA08'};MCHP.module.ADC0(1).pin.X6.Rx_idx=8;MCHP.module.ADC0(1).pin.X6.ABCD=1;MCHP.module.ADC0(1).pin.Y6.txt={ 'PA08'};MCHP.module.ADC0(1).pin.Y6.Rx_idx=8;MCHP.module.ADC0(1).pin.Y6.ABCD=1;MCHP.module.ADC0(1).pin.X7.txt={ 'PA09'};MCHP.module.ADC0(1).pin.X7.Rx_idx=9;MCHP.module.ADC0(1).pin.X7.ABCD=1;MCHP.module.ADC0(1).pin.Y7.txt={ 'PA09'};MCHP.module.ADC0(1).pin.Y7.Rx_idx=9;MCHP.module.ADC0(1).pin.Y7.ABCD=1;MCHP.module.ADC0(1).pin.X8.txt={ 'PA10'};MCHP.module.ADC0(1).pin.X8.Rx_idx=10;MCHP.module.ADC0(1).pin.X8.ABCD=1;MCHP.module.ADC0(1).pin.Y8.txt={ 'PA10'};MCHP.module.ADC0(1).pin.Y8.Rx_idx=10;MCHP.module.ADC0(1).pin.Y8.ABCD=1;MCHP.module.ADC0(1).pin.X9.txt={ 'PA11'};MCHP.module.ADC0(1).pin.X9.Rx_idx=11;MCHP.module.ADC0(1).pin.X9.ABCD=1;MCHP.module.ADC0(1).pin.Y9.txt={ 'PA11'};MCHP.module.ADC0(1).pin.Y9.Rx_idx=11;MCHP.module.ADC0(1).pin.Y9.ABCD=1;MCHP.module.ADC0(1).pin.X10.txt={ 'PA16'};MCHP.module.ADC0(1).pin.X10.Rx_idx=16;MCHP.module.ADC0(1).pin.X10.ABCD=1;MCHP.module.ADC0(1).pin.Y10.txt={ 'PA16'};MCHP.module.ADC0(1).pin.Y10.Rx_idx=16;MCHP.module.ADC0(1).pin.Y10.ABCD=1;MCHP.module.ADC0(1).pin.X11.txt={ 'PA17'};MCHP.module.ADC0(1).pin.X11.Rx_idx=17;MCHP.module.ADC0(1).pin.X11.ABCD=1;MCHP.module.ADC0(1).pin.Y11.txt={ 'PA17'};MCHP.module.ADC0(1).pin.Y11.Rx_idx=17;MCHP.module.ADC0(1).pin.Y11.ABCD=1;MCHP.module.ADC0(1).pin.X12.txt={ 'PA18'};MCHP.module.ADC0(1).pin.X12.Rx_idx=18;MCHP.module.ADC0(1).pin.X12.ABCD=1;MCHP.module.ADC0(1).pin.Y12.txt={ 'PA18'};MCHP.module.ADC0(1).pin.Y12.Rx_idx=18;MCHP.module.ADC0(1).pin.Y12.ABCD=1;MCHP.module.ADC0(1).pin.X13.txt={ 'PA19'};MCHP.module.ADC0(1).pin.X13.Rx_idx=19;MCHP.module.ADC0(1).pin.X13.ABCD=1;MCHP.module.ADC0(1).pin.Y13.txt={ 'PA19'};MCHP.module.ADC0(1).pin.Y13.Rx_idx=19;MCHP.module.ADC0(1).pin.Y13.ABCD=1;MCHP.module.ADC0(1).pin.X14.txt={ 'PA20'};MCHP.module.ADC0(1).pin.X14.Rx_idx=20;MCHP.module.ADC0(1).pin.X14.ABCD=1;MCHP.module.ADC0(1).pin.Y14.txt={ 'PA20'};MCHP.module.ADC0(1).pin.Y14.Rx_idx=20;MCHP.module.ADC0(1).pin.Y14.ABCD=1;MCHP.module.ADC0(1).pin.X15.txt={ 'PA21'};MCHP.module.ADC0(1).pin.X15.Rx_idx=21;MCHP.module.ADC0(1).pin.X15.ABCD=1;MCHP.module.ADC0(1).pin.Y15.txt={ 'PA21'};MCHP.module.ADC0(1).pin.Y15.Rx_idx=21;MCHP.module.ADC0(1).pin.Y15.ABCD=1;MCHP.module.ADC0(1).pin.X16.txt={ 'PA22'};MCHP.module.ADC0(1).pin.X16.Rx_idx=22;MCHP.module.ADC0(1).pin.X16.ABCD=1;MCHP.module.ADC0(1).pin.Y16.txt={ 'PA22'};MCHP.module.ADC0(1).pin.Y16.Rx_idx=22;MCHP.module.ADC0(1).pin.Y16.ABCD=1;MCHP.module.ADC0(1).pin.X17.txt={ 'PA23'};MCHP.module.ADC0(1).pin.X17.Rx_idx=23;MCHP.module.ADC0(1).pin.X17.ABCD=1;MCHP.module.ADC0(1).pin.Y17.txt={ 'PA23'};MCHP.module.ADC0(1).pin.Y17.Rx_idx=23;MCHP.module.ADC0(1).pin.Y17.ABCD=1;MCHP.module.ADC0(1).pin.X18.txt={ 'PA27'};MCHP.module.ADC0(1).pin.X18.Rx_idx=27;MCHP.module.ADC0(1).pin.X18.ABCD=1;MCHP.module.ADC0(1).pin.Y18.txt={ 'PA27'};MCHP.module.ADC0(1).pin.Y18.Rx_idx=27;MCHP.module.ADC0(1).pin.Y18.ABCD=1;MCHP.module.ADC0(1).pin.X19.txt={ 'PA30'};MCHP.module.ADC0(1).pin.X19.Rx_idx=30;MCHP.module.ADC0(1).pin.X19.ABCD=1;MCHP.module.ADC0(1).pin.Y19.txt={ 'PA30'};MCHP.module.ADC0(1).pin.Y19.Rx_idx=30;MCHP.module.ADC0(1).pin.Y19.ABCD=1;MCHP.module.ADC0(1).pin.X20.txt={ 'PB02'};MCHP.module.ADC0(1).pin.X20.Rx_idx=34;MCHP.module.ADC0(1).pin.X20.ABCD=1;MCHP.module.ADC0(1).pin.Y20.txt={ 'PB02'};MCHP.module.ADC0(1).pin.Y20.Rx_idx=34;MCHP.module.ADC0(1).pin.Y20.ABCD=1;MCHP.module.ADC0(1).pin.X21.txt={ 'PB03'};MCHP.module.ADC0(1).pin.X21.Rx_idx=35;MCHP.module.ADC0(1).pin.X21.ABCD=1;MCHP.module.ADC0(1).pin.Y21.txt={ 'PB03'};MCHP.module.ADC0(1).pin.Y21.Rx_idx=35;MCHP.module.ADC0(1).pin.Y21.ABCD=1;MCHP.module.ADC0(1).pin.X22.txt={ 'PB04'};MCHP.module.ADC0(1).pin.X22.Rx_idx=36;MCHP.module.ADC0(1).pin.X22.ABCD=1;MCHP.module.ADC0(1).pin.Y22.txt={ 'PB04'};MCHP.module.ADC0(1).pin.Y22.Rx_idx=36;MCHP.module.ADC0(1).pin.Y22.ABCD=1;MCHP.module.ADC0(1).pin.X23.txt={ 'PB05'};MCHP.module.ADC0(1).pin.X23.Rx_idx=37;MCHP.module.ADC0(1).pin.X23.ABCD=1;MCHP.module.ADC0(1).pin.Y23.txt={ 'PB05'};MCHP.module.ADC0(1).pin.Y23.Rx_idx=37;MCHP.module.ADC0(1).pin.Y23.ABCD=1;MCHP.module.ADC0(1).pin.X24.txt={ 'PB06'};MCHP.module.ADC0(1).pin.X24.Rx_idx=38;MCHP.module.ADC0(1).pin.X24.ABCD=1;MCHP.module.ADC0(1).pin.Y24.txt={ 'PB06'};MCHP.module.ADC0(1).pin.Y24.Rx_idx=38;MCHP.module.ADC0(1).pin.Y24.ABCD=1;MCHP.module.ADC0(1).pin.X25.txt={ 'PB07'};MCHP.module.ADC0(1).pin.X25.Rx_idx=39;MCHP.module.ADC0(1).pin.X25.ABCD=1;MCHP.module.ADC0(1).pin.Y25.txt={ 'PB07'};MCHP.module.ADC0(1).pin.Y25.Rx_idx=39;MCHP.module.ADC0(1).pin.Y25.ABCD=1;MCHP.module.ADC0(1).pin.X26.txt={ 'PB12'};MCHP.module.ADC0(1).pin.X26.Rx_idx=44;MCHP.module.ADC0(1).pin.X26.ABCD=1;MCHP.module.ADC0(1).pin.Y26.txt={ 'PB12'};MCHP.module.ADC0(1).pin.Y26.Rx_idx=44;MCHP.module.ADC0(1).pin.Y26.ABCD=1;MCHP.module.ADC0(1).pin.X27.txt={ 'PB13'};MCHP.module.ADC0(1).pin.X27.Rx_idx=45;MCHP.module.ADC0(1).pin.X27.ABCD=1;MCHP.module.ADC0(1).pin.Y27.txt={ 'PB13'};MCHP.module.ADC0(1).pin.Y27.Rx_idx=45;MCHP.module.ADC0(1).pin.Y27.ABCD=1;MCHP.module.ADC0(1).pin.X28.txt={ 'PB14'};MCHP.module.ADC0(1).pin.X28.Rx_idx=46;MCHP.module.ADC0(1).pin.X28.ABCD=1;MCHP.module.ADC0(1).pin.Y28.txt={ 'PB14'};MCHP.module.ADC0(1).pin.Y28.Rx_idx=46;MCHP.module.ADC0(1).pin.Y28.ABCD=1;MCHP.module.ADC0(1).pin.X29.txt={ 'PB15'};MCHP.module.ADC0(1).pin.X29.Rx_idx=47;MCHP.module.ADC0(1).pin.X29.ABCD=1;MCHP.module.ADC0(1).pin.Y29.txt={ 'PB15'};MCHP.module.ADC0(1).pin.Y29.Rx_idx=47;MCHP.module.ADC0(1).pin.Y29.ABCD=1;MCHP.module.ADC0(1).pin.X30.txt={ 'PB00'};MCHP.module.ADC0(1).pin.X30.Rx_idx=32;MCHP.module.ADC0(1).pin.X30.ABCD=1;MCHP.module.ADC0(1).pin.Y30.txt={ 'PB00'};MCHP.module.ADC0(1).pin.Y30.Rx_idx=32;MCHP.module.ADC0(1).pin.Y30.ABCD=1;MCHP.module.ADC0(1).pin.X31.txt={ 'PB01'};MCHP.module.ADC0(1).pin.X31.Rx_idx=33;MCHP.module.ADC0(1).pin.X31.ABCD=1;MCHP.module.ADC0(1).pin.Y31.txt={ 'PB01'};MCHP.module.ADC0(1).pin.Y31.Rx_idx=33;MCHP.module.ADC0(1).pin.Y31.ABCD=1;MCHP.module.ADC0(1).pin.VREFA.txt={ 'PA03'};MCHP.module.ADC0(1).pin.VREFA.Rx_idx=3;MCHP.module.ADC0(1).pin.VREFA.ABCD=1;MCHP.module.ADC0(1).pin.VREFB.txt={ 'PA04'};MCHP.module.ADC0(1).pin.VREFB.Rx_idx=4;MCHP.module.ADC0(1).pin.VREFB.ABCD=1;MCHP.module.ADC0(1).pin.VREFC.txt={ 'PA06'};MCHP.module.ADC0(1).pin.VREFC.Rx_idx=6;MCHP.module.ADC0(1).pin.VREFC.ABCD=1;MCHP.module.ADC0(2).PID=119;MCHP.module.ADC0(2).vector='ADC0_RESRDY';MCHP.module.ADC0(2).pin=reshape(MCHP_Fun.Hex2num('[]'),0,0);MCHP.module.ADC1(1).PID=120;MCHP.module.ADC1(1).vector='ADC1_OTHER';MCHP.module.ADC1(1).pin.AIN0.txt={ 'PB08'};MCHP.module.ADC1(1).pin.AIN0.Rx_idx=40;MCHP.module.ADC1(1).pin.AIN0.ABCD=1;MCHP.module.ADC1(1).pin.AIN1.txt={ 'PB09'};MCHP.module.ADC1(1).pin.AIN1.Rx_idx=41;MCHP.module.ADC1(1).pin.AIN1.ABCD=1;MCHP.module.ADC1(1).pin.AIN2.txt={ 'PA08'};MCHP.module.ADC1(1).pin.AIN2.Rx_idx=8;MCHP.module.ADC1(1).pin.AIN2.ABCD=1;MCHP.module.ADC1(1).pin.AIN3.txt={ 'PA09'};MCHP.module.ADC1(1).pin.AIN3.Rx_idx=9;MCHP.module.ADC1(1).pin.AIN3.ABCD=1;MCHP.module.ADC1(1).pin.AIN4.txt={ 'PC02'};MCHP.module.ADC1(1).pin.AIN4.Rx_idx=66;MCHP.module.ADC1(1).pin.AIN4.ABCD=1;MCHP.module.ADC1(1).pin.AIN5.txt={ 'PC03'};MCHP.module.ADC1(1).pin.AIN5.Rx_idx=67;MCHP.module.ADC1(1).pin.AIN5.ABCD=1;MCHP.module.ADC1(1).pin.AIN6.txt={ 'PB04'};MCHP.module.ADC1(1).pin.AIN6.Rx_idx=36;MCHP.module.ADC1(1).pin.AIN6.ABCD=1;MCHP.module.ADC1(1).pin.AIN7.txt={ 'PB05'};MCHP.module.ADC1(1).pin.AIN7.Rx_idx=37;MCHP.module.ADC1(1).pin.AIN7.ABCD=1;MCHP.module.ADC1(1).pin.AIN8.txt={ 'PB06'};MCHP.module.ADC1(1).pin.AIN8.Rx_idx=38;MCHP.module.ADC1(1).pin.AIN8.ABCD=1;MCHP.module.ADC1(1).pin.AIN9.txt={ 'PB07'};MCHP.module.ADC1(1).pin.AIN9.Rx_idx=39;MCHP.module.ADC1(1).pin.AIN9.ABCD=1;MCHP.module.ADC1(1).pin.AIN10.txt={ 'PC00'};MCHP.module.ADC1(1).pin.AIN10.Rx_idx=64;MCHP.module.ADC1(1).pin.AIN10.ABCD=1;MCHP.module.ADC1(1).pin.AIN11.txt={ 'PC01'};MCHP.module.ADC1(1).pin.AIN11.Rx_idx=65;MCHP.module.ADC1(1).pin.AIN11.ABCD=1;MCHP.module.ADC1(1).pin.AIN12.txt={ 'PC30'};MCHP.module.ADC1(1).pin.AIN12.Rx_idx=94;MCHP.module.ADC1(1).pin.AIN12.ABCD=1;MCHP.module.ADC1(1).pin.AIN13.txt={ 'PC31'};MCHP.module.ADC1(1).pin.AIN13.Rx_idx=95;MCHP.module.ADC1(1).pin.AIN13.ABCD=1;MCHP.module.ADC1(1).pin.AIN14.txt={ 'PD00'};MCHP.module.ADC1(1).pin.AIN14.Rx_idx=96;MCHP.module.ADC1(1).pin.AIN14.ABCD=1;MCHP.module.ADC1(1).pin.AIN15.txt={ 'PD01'};MCHP.module.ADC1(1).pin.AIN15.Rx_idx=97;MCHP.module.ADC1(1).pin.AIN15.ABCD=1;MCHP.module.ADC1(2).PID=121;MCHP.module.ADC1(2).vector='ADC1_RESRDY';MCHP.module.ADC1(2).pin=reshape(MCHP_Fun.Hex2num('[]'),0,0);MCHP.module.AC.PID=122;MCHP.module.AC.vector='AC';MCHP.module.AC.pin.AIN0.txt={ 'PA04'};MCHP.module.AC.pin.AIN0.Rx_idx=4;MCHP.module.AC.pin.AIN0.ABCD=1;MCHP.module.AC.pin.AIN1.txt={ 'PA05'};MCHP.module.AC.pin.AIN1.Rx_idx=5;MCHP.module.AC.pin.AIN1.ABCD=1;MCHP.module.AC.pin.AIN2.txt={ 'PA06'};MCHP.module.AC.pin.AIN2.Rx_idx=6;MCHP.module.AC.pin.AIN2.ABCD=1;MCHP.module.AC.pin.AIN3.txt={ 'PA07'};MCHP.module.AC.pin.AIN3.Rx_idx=7;MCHP.module.AC.pin.AIN3.ABCD=1;MCHP.module.AC.pin.CMP0.txt=reshape({ 'PA12','PA18','PB24'},1,3);MCHP.module.AC.pin.CMP0.Rx_idx=reshape([12 18 56],1,3);MCHP.module.AC.pin.CMP0.ABCD=reshape([12 12 12],1,3);MCHP.module.AC.pin.CMP1.txt=reshape({ 'PA13','PA19','PB25'},1,3);MCHP.module.AC.pin.CMP1.Rx_idx=reshape([13 19 57],1,3);MCHP.module.AC.pin.CMP1.ABCD=reshape([12 12 12],1,3);MCHP.module.DAC(1).PID=123;MCHP.module.DAC(1).vector='DAC_OTHER';MCHP.module.DAC(1).pin.VOUT0.txt={ 'PA02'};MCHP.module.DAC(1).pin.VOUT0.Rx_idx=2;MCHP.module.DAC(1).pin.VOUT0.ABCD=1;MCHP.module.DAC(1).pin.VOUT1.txt={ 'PA05'};MCHP.module.DAC(1).pin.VOUT1.Rx_idx=5;MCHP.module.DAC(1).pin.VOUT1.ABCD=1;MCHP.module.DAC(2).PID=124;MCHP.module.DAC(2).vector='DAC_EMPTY_0';MCHP.module.DAC(2).pin=reshape(MCHP_Fun.Hex2num('[]'),0,0);MCHP.module.DAC(3).PID=125;MCHP.module.DAC(3).vector='DAC_EMPTY_1';MCHP.module.DAC(3).pin=reshape(MCHP_Fun.Hex2num('[]'),0,0);MCHP.module.DAC(4).PID=126;MCHP.module.DAC(4).vector='DAC_RESRDY_0';MCHP.module.DAC(4).pin=reshape(MCHP_Fun.Hex2num('[]'),0,0);MCHP.module.DAC(5).PID=127;MCHP.module.DAC(5).vector='DAC_RESRDY_1';MCHP.module.DAC(5).pin=reshape(MCHP_Fun.Hex2num('[]'),0,0);MCHP.module.I2S.PID=128;MCHP.module.I2S.vector='I2S';MCHP.module.I2S.pin.FS0.txt=reshape({ 'PA09','PA20'},1,2);MCHP.module.I2S.pin.FS0.Rx_idx=reshape([9 20],1,2);MCHP.module.I2S.pin.FS0.ABCD=reshape([9 9],1,2);MCHP.module.I2S.pin.FS1.txt=reshape({ 'PA23','PB11'},1,2);MCHP.module.I2S.pin.FS1.Rx_idx=reshape([23 43],1,2);MCHP.module.I2S.pin.FS1.ABCD=reshape([9 9],1,2);MCHP.module.I2S.pin.MCK0.txt=reshape({ 'PA08','PB17'},1,2);MCHP.module.I2S.pin.MCK0.Rx_idx=reshape([8 49],1,2);MCHP.module.I2S.pin.MCK0.ABCD=reshape([9 9],1,2);MCHP.module.I2S.pin.MCK1.txt=reshape({ 'PB29','PB13'},1,2);MCHP.module.I2S.pin.MCK1.Rx_idx=reshape([61 45],1,2);MCHP.module.I2S.pin.MCK1.ABCD=reshape([9 9],1,2);MCHP.module.I2S.pin.SCK0.txt=reshape({ 'PA10','PB16'},1,2);MCHP.module.I2S.pin.SCK0.Rx_idx=reshape([10 48],1,2);MCHP.module.I2S.pin.SCK0.ABCD=reshape([9 9],1,2);MCHP.module.I2S.pin.SCK1.txt=reshape({ 'PB28','PB12'},1,2);MCHP.module.I2S.pin.SCK1.Rx_idx=reshape([60 44],1,2);MCHP.module.I2S.pin.SCK1.ABCD=reshape([9 9],1,2);MCHP.module.I2S.pin.SDI.txt=reshape({ 'PA22','PB10'},1,2);MCHP.module.I2S.pin.SDI.Rx_idx=reshape([22 42],1,2);MCHP.module.I2S.pin.SDI.ABCD=reshape([9 9],1,2);MCHP.module.I2S.pin.SDO.txt=reshape({ 'PA11','PA21'},1,2);MCHP.module.I2S.pin.SDO.Rx_idx=reshape([11 21],1,2);MCHP.module.I2S.pin.SDO.ABCD=reshape([9 9],1,2);MCHP.module.PCC.PID=129;MCHP.module.PCC.vector='PCC';MCHP.module.PCC.pin.CLK.txt={ 'PA14'};MCHP.module.PCC.pin.CLK.Rx_idx=14;MCHP.module.PCC.pin.CLK.ABCD=10;MCHP.module.PCC.pin.DATA0.txt={ 'PA16'};MCHP.module.PCC.pin.DATA0.Rx_idx=16;MCHP.module.PCC.pin.DATA0.ABCD=10;MCHP.module.PCC.pin.DATA1.txt={ 'PA17'};MCHP.module.PCC.pin.DATA1.Rx_idx=17;MCHP.module.PCC.pin.DATA1.ABCD=10;MCHP.module.PCC.pin.DATA2.txt={ 'PA18'};MCHP.module.PCC.pin.DATA2.Rx_idx=18;MCHP.module.PCC.pin.DATA2.ABCD=10;MCHP.module.PCC.pin.DATA3.txt={ 'PA19'};MCHP.module.PCC.pin.DATA3.Rx_idx=19;MCHP.module.PCC.pin.DATA3.ABCD=10;MCHP.module.PCC.pin.DATA4.txt={ 'PA20'};MCHP.module.PCC.pin.DATA4.Rx_idx=20;MCHP.module.PCC.pin.DATA4.ABCD=10;MCHP.module.PCC.pin.DATA5.txt={ 'PA21'};MCHP.module.PCC.pin.DATA5.Rx_idx=21;MCHP.module.PCC.pin.DATA5.ABCD=10;MCHP.module.PCC.pin.DATA6.txt={ 'PA22'};MCHP.module.PCC.pin.DATA6.Rx_idx=22;MCHP.module.PCC.pin.DATA6.ABCD=10;MCHP.module.PCC.pin.DATA7.txt={ 'PA23'};MCHP.module.PCC.pin.DATA7.Rx_idx=23;MCHP.module.PCC.pin.DATA7.ABCD=10;MCHP.module.PCC.pin.DATA8.txt={ 'PB14'};MCHP.module.PCC.pin.DATA8.Rx_idx=46;MCHP.module.PCC.pin.DATA8.ABCD=10;MCHP.module.PCC.pin.DATA9.txt={ 'PB15'};MCHP.module.PCC.pin.DATA9.Rx_idx=47;MCHP.module.PCC.pin.DATA9.ABCD=10;MCHP.module.PCC.pin.DATA10.txt={ 'PC12'};MCHP.module.PCC.pin.DATA10.Rx_idx=76;MCHP.module.PCC.pin.DATA10.ABCD=10;MCHP.module.PCC.pin.DATA11.txt={ 'PC13'};MCHP.module.PCC.pin.DATA11.Rx_idx=77;MCHP.module.PCC.pin.DATA11.ABCD=10;MCHP.module.PCC.pin.DATA12.txt={ 'PC14'};MCHP.module.PCC.pin.DATA12.Rx_idx=78;MCHP.module.PCC.pin.DATA12.ABCD=10;MCHP.module.PCC.pin.DATA13.txt={ 'PC15'};MCHP.module.PCC.pin.DATA13.Rx_idx=79;MCHP.module.PCC.pin.DATA13.ABCD=10;MCHP.module.PCC.pin.DEN1.txt={ 'PA12'};MCHP.module.PCC.pin.DEN1.Rx_idx=12;MCHP.module.PCC.pin.DEN1.ABCD=10;MCHP.module.PCC.pin.DEN2.txt={ 'PA13'};MCHP.module.PCC.pin.DEN2.Rx_idx=13;MCHP.module.PCC.pin.DEN2.ABCD=10;MCHP.module.AES.PID=130;MCHP.module.AES.vector='AES';MCHP.module.TRNG.PID=131;MCHP.module.TRNG.vector='TRNG';MCHP.module.ICM.PID=132;MCHP.module.ICM.vector='ICM';MCHP.module.PUKCC.PID=133;MCHP.module.PUKCC.vector='PUKCC';MCHP.module.QSPI.PID=134;MCHP.module.QSPI.vector='QSPI';MCHP.module.QSPI.pin.CS.txt={ 'PB11'};MCHP.module.QSPI.pin.CS.Rx_idx=43;MCHP.module.QSPI.pin.CS.ABCD=7;MCHP.module.QSPI.pin.DATA0.txt={ 'PA08'};MCHP.module.QSPI.pin.DATA0.Rx_idx=8;MCHP.module.QSPI.pin.DATA0.ABCD=7;MCHP.module.QSPI.pin.DATA1.txt={ 'PA09'};MCHP.module.QSPI.pin.DATA1.Rx_idx=9;MCHP.module.QSPI.pin.DATA1.ABCD=7;MCHP.module.QSPI.pin.DATA2.txt={ 'PA10'};MCHP.module.QSPI.pin.DATA2.Rx_idx=10;MCHP.module.QSPI.pin.DATA2.ABCD=7;MCHP.module.QSPI.pin.DATA3.txt={ 'PA11'};MCHP.module.QSPI.pin.DATA3.Rx_idx=11;MCHP.module.QSPI.pin.DATA3.ABCD=7;MCHP.module.QSPI.pin.SCK.txt={ 'PB10'};MCHP.module.QSPI.pin.SCK.Rx_idx=42;MCHP.module.QSPI.pin.SCK.ABCD=7;MCHP.module.SDHC0.PID=135;MCHP.module.SDHC0.vector='SDHC0';MCHP.module.SDHC0.pin.SDCD.txt=reshape({ 'PA06','PA12','PB12','PC06'},1,4);MCHP.module.SDHC0.pin.SDCD.Rx_idx=reshape([6 12 44 70],1,4);MCHP.module.SDHC0.pin.SDCD.ABCD=reshape([8 8 8 8],1,4);MCHP.module.SDHC0.pin.SDCK.txt={ 'PB11'};MCHP.module.SDHC0.pin.SDCK.Rx_idx=43;MCHP.module.SDHC0.pin.SDCK.ABCD=8;MCHP.module.SDHC0.pin.SDCMD.txt={ 'PA08'};MCHP.module.SDHC0.pin.SDCMD.Rx_idx=8;MCHP.module.SDHC0.pin.SDCMD.ABCD=8;MCHP.module.SDHC0.pin.SDDAT0.txt={ 'PA09'};MCHP.module.SDHC0.pin.SDDAT0.Rx_idx=9;MCHP.module.SDHC0.pin.SDDAT0.ABCD=8;MCHP.module.SDHC0.pin.SDDAT1.txt={ 'PA10'};MCHP.module.SDHC0.pin.SDDAT1.Rx_idx=10;MCHP.module.SDHC0.pin.SDDAT1.ABCD=8;MCHP.module.SDHC0.pin.SDDAT2.txt={ 'PA11'};MCHP.module.SDHC0.pin.SDDAT2.Rx_idx=11;MCHP.module.SDHC0.pin.SDDAT2.ABCD=8;MCHP.module.SDHC0.pin.SDDAT3.txt={ 'PB10'};MCHP.module.SDHC0.pin.SDDAT3.Rx_idx=42;MCHP.module.SDHC0.pin.SDDAT3.ABCD=8;MCHP.module.SDHC0.pin.SDWP.txt=reshape({ 'PA07','PA13','PB13','PC07'},1,4);MCHP.module.SDHC0.pin.SDWP.Rx_idx=reshape([7 13 45 71],1,4);MCHP.module.SDHC0.pin.SDWP.ABCD=reshape([8 8 8 8],1,4);MCHP.module.SDHC1.PID=136;MCHP.module.SDHC1.vector='SDHC1';MCHP.module.SDHC1.pin.SDCD.txt=reshape({ 'PB16','PC20','PD20'},1,3);MCHP.module.SDHC1.pin.SDCD.Rx_idx=reshape([48 84 116],1,3);MCHP.module.SDHC1.pin.SDCD.ABCD=reshape([8 8 8],1,3);MCHP.module.SDHC1.pin.SDCK.txt={ 'PA21'};MCHP.module.SDHC1.pin.SDCK.Rx_idx=21;MCHP.module.SDHC1.pin.SDCK.ABCD=8;MCHP.module.SDHC1.pin.SDCMD.txt={ 'PA20'};MCHP.module.SDHC1.pin.SDCMD.Rx_idx=20;MCHP.module.SDHC1.pin.SDCMD.ABCD=8;MCHP.module.SDHC1.pin.SDDAT0.txt={ 'PB18'};MCHP.module.SDHC1.pin.SDDAT0.Rx_idx=50;MCHP.module.SDHC1.pin.SDDAT0.ABCD=8;MCHP.module.SDHC1.pin.SDDAT1.txt={ 'PB19'};MCHP.module.SDHC1.pin.SDDAT1.Rx_idx=51;MCHP.module.SDHC1.pin.SDDAT1.ABCD=8;MCHP.module.SDHC1.pin.SDDAT2.txt={ 'PB20'};MCHP.module.SDHC1.pin.SDDAT2.Rx_idx=52;MCHP.module.SDHC1.pin.SDDAT2.ABCD=8;MCHP.module.SDHC1.pin.SDDAT3.txt={ 'PB21'};MCHP.module.SDHC1.pin.SDDAT3.Rx_idx=53;MCHP.module.SDHC1.pin.SDDAT3.ABCD=8;MCHP.module.SDHC1.pin.SDWP.txt=reshape({ 'PB17','PC21','PD21'},1,3);MCHP.module.SDHC1.pin.SDWP.Rx_idx=reshape([49 85 117],1,3);MCHP.module.SDHC1.pin.SDWP.ABCD=reshape([8 8 8],1,3);MCHP.module.CCL.pin.IN0.txt=reshape({ 'PA04','PA16','PB22'},1,3);MCHP.module.CCL.pin.IN0.Rx_idx=reshape([4 16 54],1,3);MCHP.module.CCL.pin.IN0.ABCD=reshape([13 13 13],1,3);MCHP.module.CCL.pin.IN1.txt=reshape({ 'PA05','PA17','PB00'},1,3);MCHP.module.CCL.pin.IN1.Rx_idx=reshape([5 17 32],1,3);MCHP.module.CCL.pin.IN1.ABCD=reshape([13 13 13],1,3);MCHP.module.CCL.pin.IN2.txt=reshape({ 'PA06','PA18','PB01'},1,3);MCHP.module.CCL.pin.IN2.Rx_idx=reshape([6 18 33],1,3);MCHP.module.CCL.pin.IN2.ABCD=reshape([13 13 13],1,3);MCHP.module.CCL.pin.IN3.txt=reshape({ 'PA08','PA30'},1,2);MCHP.module.CCL.pin.IN3.Rx_idx=reshape([8 30],1,2);MCHP.module.CCL.pin.IN3.ABCD=reshape([13 13],1,2);MCHP.module.CCL.pin.IN4.txt=reshape({ 'PA09','PC27'},1,2);MCHP.module.CCL.pin.IN4.Rx_idx=reshape([9 91],1,2);MCHP.module.CCL.pin.IN4.ABCD=reshape([13 13],1,2);MCHP.module.CCL.pin.IN5.txt=reshape({ 'PA10','PC28'},1,2);MCHP.module.CCL.pin.IN5.Rx_idx=reshape([10 92],1,2);MCHP.module.CCL.pin.IN5.ABCD=reshape([13 13],1,2);MCHP.module.CCL.pin.IN6.txt=reshape({ 'PA22','PB06'},1,2);MCHP.module.CCL.pin.IN6.Rx_idx=reshape([22 38],1,2);MCHP.module.CCL.pin.IN6.ABCD=reshape([13 13],1,2);MCHP.module.CCL.pin.IN7.txt=reshape({ 'PA23','PB07'},1,2);MCHP.module.CCL.pin.IN7.Rx_idx=reshape([23 39],1,2);MCHP.module.CCL.pin.IN7.ABCD=reshape([13 13],1,2);MCHP.module.CCL.pin.IN8.txt=reshape({ 'PA24','PB08'},1,2);MCHP.module.CCL.pin.IN8.Rx_idx=reshape([24 40],1,2);MCHP.module.CCL.pin.IN8.ABCD=reshape([13 13],1,2);MCHP.module.CCL.pin.IN9.txt=reshape({ 'PB14','PC20'},1,2);MCHP.module.CCL.pin.IN9.Rx_idx=reshape([46 84],1,2);MCHP.module.CCL.pin.IN9.ABCD=reshape([13 13],1,2);MCHP.module.CCL.pin.IN10.txt=reshape({ 'PB15','PC21'},1,2);MCHP.module.CCL.pin.IN10.Rx_idx=reshape([47 85],1,2);MCHP.module.CCL.pin.IN10.ABCD=reshape([13 13],1,2);MCHP.module.CCL.pin.IN11.txt=reshape({ 'PB10','PB16'},1,2);MCHP.module.CCL.pin.IN11.Rx_idx=reshape([42 48],1,2);MCHP.module.CCL.pin.IN11.ABCD=reshape([13 13],1,2);MCHP.module.CCL.pin.OUT0.txt=reshape({ 'PA07','PA19','PB02','PB23'},1,4);MCHP.module.CCL.pin.OUT0.Rx_idx=reshape([7 19 34 55],1,4);MCHP.module.CCL.pin.OUT0.ABCD=reshape([13 13 13 13],1,4);MCHP.module.CCL.pin.OUT1.txt=reshape({ 'PA11','PA31','PB11'},1,3);MCHP.module.CCL.pin.OUT1.Rx_idx=reshape([11 31 43],1,3);MCHP.module.CCL.pin.OUT1.ABCD=reshape([13 13 13],1,3);MCHP.module.CCL.pin.OUT2.txt=reshape({ 'PA25','PB09'},1,2);MCHP.module.CCL.pin.OUT2.Rx_idx=reshape([25 41],1,2);MCHP.module.CCL.pin.OUT2.ABCD=reshape([13 13],1,2);MCHP.module.CCL.pin.OUT3.txt={ 'PB17'};MCHP.module.CCL.pin.OUT3.Rx_idx=49;MCHP.module.CCL.pin.OUT3.ABCD=13;MCHP.module.GCLK.pin.IO0.txt=reshape({ 'PA30','PB14','PA14','PB22'},1,4);MCHP.module.GCLK.pin.IO0.Rx_idx=reshape([30 46 14 54],1,4);MCHP.module.GCLK.pin.IO0.ABCD=reshape([12 12 12 12],1,4);MCHP.module.GCLK.pin.IO1.txt=reshape({ 'PB15','PA15','PB23','PA27'},1,4);MCHP.module.GCLK.pin.IO1.Rx_idx=reshape([47 15 55 27],1,4);MCHP.module.GCLK.pin.IO1.ABCD=reshape([12 12 12 12],1,4);MCHP.module.GCLK.pin.IO2.txt=reshape({ 'PA16','PB16'},1,2);MCHP.module.GCLK.pin.IO2.Rx_idx=reshape([16 48],1,2);MCHP.module.GCLK.pin.IO2.ABCD=reshape([12 12],1,2);MCHP.module.GCLK.pin.IO3.txt=reshape({ 'PA17','PB17'},1,2);MCHP.module.GCLK.pin.IO3.Rx_idx=reshape([17 49],1,2);MCHP.module.GCLK.pin.IO3.ABCD=reshape([12 12],1,2);MCHP.module.GCLK.pin.IO4.txt=reshape({ 'PA10','PB10','PB18'},1,3);MCHP.module.GCLK.pin.IO4.Rx_idx=reshape([10 42 50],1,3);MCHP.module.GCLK.pin.IO4.ABCD=reshape([12 12 12],1,3);MCHP.module.GCLK.pin.IO5.txt=reshape({ 'PA11','PB11','PB19'},1,3);MCHP.module.GCLK.pin.IO5.Rx_idx=reshape([11 43 51],1,3);MCHP.module.GCLK.pin.IO5.ABCD=reshape([12 12 12],1,3);MCHP.module.GCLK.pin.IO6.txt=reshape({ 'PB12','PB20'},1,2);MCHP.module.GCLK.pin.IO6.Rx_idx=reshape([44 52],1,2);MCHP.module.GCLK.pin.IO6.ABCD=reshape([12 12],1,2);MCHP.module.GCLK.pin.IO7.txt=reshape({ 'PB13','PB21'},1,2);MCHP.module.GCLK.pin.IO7.Rx_idx=reshape([45 53],1,2);MCHP.module.GCLK.pin.IO7.ABCD=reshape([12 12],1,2);MCHP.module.TPIU.pin.TRACECLK.txt={ 'PC27'};MCHP.module.TPIU.pin.TRACECLK.Rx_idx=91;MCHP.module.TPIU.pin.TRACECLK.ABCD=7;MCHP.module.TPIU.pin.TRACED0.txt={ 'PC28'};MCHP.module.TPIU.pin.TRACED0.Rx_idx=92;MCHP.module.TPIU.pin.TRACED0.ABCD=7;MCHP.module.TPIU.pin.TRACED1.txt={ 'PC26'};MCHP.module.TPIU.pin.TRACED1.Rx_idx=90;MCHP.module.TPIU.pin.TRACED1.ABCD=7;MCHP.module.TPIU.pin.TRACED2.txt={ 'PC25'};MCHP.module.TPIU.pin.TRACED2.Rx_idx=89;MCHP.module.TPIU.pin.TRACED2.ABCD=7;MCHP.module.TPIU.pin.TRACED3.txt={ 'PC24'};MCHP.module.TPIU.pin.TRACED3.Rx_idx=88;MCHP.module.TPIU.pin.TRACED3.ABCD=7;MCHP.module.FUSES.reglist=reshape({ 'USER_WORD_0','USER_WORD_1','USER_WORD_2'},1,3);MCHP.module.FUSES.reg.USER_WORD_0.caption='USER Page Word 0';MCHP.module.FUSES.reg.USER_WORD_0.bitfieldList=reshape({ 'BOD33_DIS','BOD33USERLEVEL','BOD33_ACTION','BOD33_HYST','NVMCTRL_BOOTPROT'},1,5);MCHP.module.FUSES.reg.USER_WORD_0.BOD33_DIS.mask=2;MCHP.module.FUSES.reg.USER_WORD_0.BOD33_DIS.choice=reshape({ 'CLEAR','SET'},1,2);MCHP.module.FUSES.reg.USER_WORD_0.BOD33_DIS.choiceCaption=reshape({ 'clear','set'},1,2);MCHP.module.FUSES.reg.USER_WORD_0.BOD33_DIS.choiceDefault='SET';MCHP.module.FUSES.reg.USER_WORD_0.BOD33USERLEVEL.mask=256;MCHP.module.FUSES.reg.USER_WORD_0.BOD33USERLEVEL.choice={};MCHP.module.FUSES.reg.USER_WORD_0.BOD33USERLEVEL.choiceCaption={ 'range in [0 - 255]'};MCHP.module.FUSES.reg.USER_WORD_0.BOD33USERLEVEL.choiceDefault='0xFF';MCHP.module.FUSES.reg.USER_WORD_0.BOD33_ACTION.mask=4;MCHP.module.FUSES.reg.USER_WORD_0.BOD33_ACTION.choice=reshape({ 'NONE','RESET','INT','BKUP'},1,4);MCHP.module.FUSES.reg.USER_WORD_0.BOD33_ACTION.choiceCaption=reshape({ 'No action','The BOD33 generates a reset','The BOD33 generates an interrupt','The BOD33 puts the device in backup sleep mode'},1,4);MCHP.module.FUSES.reg.USER_WORD_0.BOD33_ACTION.choiceDefault='NONE';MCHP.module.FUSES.reg.USER_WORD_0.BOD33_HYST.mask=16;MCHP.module.FUSES.reg.USER_WORD_0.BOD33_HYST.choice=reshape({ '0','1','2','3','4','5','6','7','8','9','A','B','C','D','E','F','10'},1,17);MCHP.module.FUSES.reg.USER_WORD_0.BOD33_HYST.choiceCaption=reshape({ '0','1','2','3','4','5','6','7','8','9','A','B','C','D','E','F','10'},1,17);MCHP.module.FUSES.reg.USER_WORD_0.BOD33_HYST.choiceDefault='0xF';MCHP.module.FUSES.reg.USER_WORD_0.NVMCTRL_BOOTPROT.mask=16;MCHP.module.FUSES.reg.USER_WORD_0.NVMCTRL_BOOTPROT.choice=reshape({ '0','8','16','24','32','40','48','56','64','72','80','88','96','104','112','120'},1,16);MCHP.module.FUSES.reg.USER_WORD_0.NVMCTRL_BOOTPROT.choiceCaption=reshape({ '0 kbytes','8 kbytes','16 kbytes','24 kbytes','32 kbytes','40 kbytes','48 kbytes','56 kbytes','64 kbytes','72 kbytes','80 kbytes','88 kbytes','96 kbytes','104 kbytes','112 kbytes','120 kbytes'},1,16);MCHP.module.FUSES.reg.USER_WORD_0.NVMCTRL_BOOTPROT.choiceDefault='0';MCHP.module.FUSES.reg.USER_WORD_1.caption='USER Page Word 1';MCHP.module.FUSES.reg.USER_WORD_1.bitfieldList=reshape({ 'NVMCTRL_SEESBLK','NVMCTRL_SEEPSZ','RAMECC_ECCDIS','WDT_ENABLE','WDT_ALWAYSON','WDT_PER','WDT_WINDOW','WDT_EWOFFSET','WDT_WEN'},1,9);MCHP.module.FUSES.reg.USER_WORD_1.NVMCTRL_SEESBLK.mask=16;MCHP.module.FUSES.reg.USER_WORD_1.NVMCTRL_SEESBLK.choice=reshape({ '0','1','2','3','4','5','6','7','8','9','A','B','C','D','E','F','10'},1,17);MCHP.module.FUSES.reg.USER_WORD_1.NVMCTRL_SEESBLK.choiceCaption=reshape({ '0','1','2','3','4','5','6','7','8','9','A','B','C','D','E','F','10'},1,17);MCHP.module.FUSES.reg.USER_WORD_1.NVMCTRL_SEESBLK.choiceDefault='0xF';MCHP.module.FUSES.reg.USER_WORD_1.NVMCTRL_SEEPSZ.mask=8;MCHP.module.FUSES.reg.USER_WORD_1.NVMCTRL_SEEPSZ.choice=reshape({ '0','1','2','3','4','5','6','7','8'},1,9);MCHP.module.FUSES.reg.USER_WORD_1.NVMCTRL_SEEPSZ.choiceCaption=reshape({ '0','1','2','3','4','5','6','7','8'},1,9);MCHP.module.FUSES.reg.USER_WORD_1.NVMCTRL_SEEPSZ.choiceDefault='0x7';MCHP.module.FUSES.reg.USER_WORD_1.RAMECC_ECCDIS.mask=2;MCHP.module.FUSES.reg.USER_WORD_1.RAMECC_ECCDIS.choice=reshape({ 'CLEAR','SET'},1,2);MCHP.module.FUSES.reg.USER_WORD_1.RAMECC_ECCDIS.choiceCaption=reshape({ 'clear','set'},1,2);MCHP.module.FUSES.reg.USER_WORD_1.RAMECC_ECCDIS.choiceDefault='SET';MCHP.module.FUSES.reg.USER_WORD_1.WDT_ENABLE.mask=2;MCHP.module.FUSES.reg.USER_WORD_1.WDT_ENABLE.choice=reshape({ 'CLEAR','SET'},1,2);MCHP.module.FUSES.reg.USER_WORD_1.WDT_ENABLE.choiceCaption=reshape({ 'clear','set'},1,2);MCHP.module.FUSES.reg.USER_WORD_1.WDT_ENABLE.choiceDefault='CLEAR';MCHP.module.FUSES.reg.USER_WORD_1.WDT_ALWAYSON.mask=2;MCHP.module.FUSES.reg.USER_WORD_1.WDT_ALWAYSON.choice=reshape({ 'CLEAR','SET'},1,2);MCHP.module.FUSES.reg.USER_WORD_1.WDT_ALWAYSON.choiceCaption=reshape({ 'clear','set'},1,2);MCHP.module.FUSES.reg.USER_WORD_1.WDT_ALWAYSON.choiceDefault='CLEAR';MCHP.module.FUSES.reg.USER_WORD_1.WDT_PER.mask=16;MCHP.module.FUSES.reg.USER_WORD_1.WDT_PER.choice=reshape({ 'CYC8','CYC16','CYC32','CYC64','CYC128','CYC256','CYC512','CYC1024','CYC2048','CYC4096','CYC8192','CYC16384'},1,12);MCHP.module.FUSES.reg.USER_WORD_1.WDT_PER.choiceCaption=reshape({ '8 clock cycles','16 clock cycles','32 clock cycles','64 clock cycles','128 clock cycles','256 clock cycles','512 clock cycles','1024 clock cycles','2048 clock cycles','4096 clock cycles','8192 clock cycles','16384 clock cycles'},1,12);MCHP.module.FUSES.reg.USER_WORD_1.WDT_PER.choiceDefault='CYC16384';MCHP.module.FUSES.reg.USER_WORD_1.WDT_WINDOW.mask=16;MCHP.module.FUSES.reg.USER_WORD_1.WDT_WINDOW.choice=reshape({ 'CYC8','CYC16','CYC32','CYC64','CYC128','CYC256','CYC512','CYC1024','CYC2048','CYC4096','CYC8192','CYC16384'},1,12);MCHP.module.FUSES.reg.USER_WORD_1.WDT_WINDOW.choiceCaption=reshape({ '8 clock cycles','16 clock cycles','32 clock cycles','64 clock cycles','128 clock cycles','256 clock cycles','512 clock cycles','1024 clock cycles','2048 clock cycles','4096 clock cycles','8192 clock cycles','16384 clock cycles'},1,12);MCHP.module.FUSES.reg.USER_WORD_1.WDT_WINDOW.choiceDefault='CYC16384';MCHP.module.FUSES.reg.USER_WORD_1.WDT_EWOFFSET.mask=16;MCHP.module.FUSES.reg.USER_WORD_1.WDT_EWOFFSET.choice=reshape({ 'CYC8','CYC16','CYC32','CYC64','CYC128','CYC256','CYC512','CYC1024','CYC2048','CYC4096','CYC8192','CYC16384'},1,12);MCHP.module.FUSES.reg.USER_WORD_1.WDT_EWOFFSET.choiceCaption=reshape({ '8 clock cycles','16 clock cycles','32 clock cycles','64 clock cycles','128 clock cycles','256 clock cycles','512 clock cycles','1024 clock cycles','2048 clock cycles','4096 clock cycles','8192 clock cycles','16384 clock cycles'},1,12);MCHP.module.FUSES.reg.USER_WORD_1.WDT_EWOFFSET.choiceDefault='CYC16384';MCHP.module.FUSES.reg.USER_WORD_1.WDT_WEN.mask=2;MCHP.module.FUSES.reg.USER_WORD_1.WDT_WEN.choice=reshape({ 'CLEAR','SET'},1,2);MCHP.module.FUSES.reg.USER_WORD_1.WDT_WEN.choiceCaption=reshape({ 'clear','set'},1,2);MCHP.module.FUSES.reg.USER_WORD_1.WDT_WEN.choiceDefault='CLEAR';MCHP.module.FUSES.reg.USER_WORD_2.caption='USER Page Word 2';MCHP.module.FUSES.reg.USER_WORD_2.bitfieldList={ 'NVMCTRL_REGION_LOCKS'};MCHP.module.FUSES.reg.USER_WORD_2.NVMCTRL_REGION_LOCKS.mask=MCHP_Fun.Hex2num('41F0000000000000');MCHP.module.FUSES.reg.USER_WORD_2.NVMCTRL_REGION_LOCKS.choice={};MCHP.module.FUSES.reg.USER_WORD_2.NVMCTRL_REGION_LOCKS.choiceCaption={ 'range in [0 - 4294967295]'};MCHP.module.FUSES.reg.USER_WORD_2.NVMCTRL_REGION_LOCKS.choiceDefault='0xFFFFFFFF';MCHP.modsrc.id_U2501=1;MCHP.modsrc.id_U2500=2;MCHP.modsrc.id_U2238=1;MCHP.modsrc.id_U2003=2;MCHP.modsrc.id_U2225=1;MCHP.modsrc.id_U2015=1;MCHP.modsrc.id_U2502=1;MCHP.modsrc.id_U2503=1;MCHP.modsrc.id_U2410=1;MCHP.modsrc.id_U2254=1;MCHP.modsrc.id_U2504=1;MCHP.modsrc.id_U2257=1;MCHP.modsrc.id_U2122=1;MCHP.modsrc.id_U2005=1;MCHP.modsrc.id_I7638=1;MCHP.modsrc.id_U2010=1;MCHP.modsrc.id_U2224=1;MCHP.modsrc.id_U2408=1;MCHP.modsrc.id_U2409=1;MCHP.modsrc.id_U2401=1;MCHP.modsrc.id_U2400=1;MCHP.modsrc.id_U2120=1;MCHP.modsrc.id_U2017=1;MCHP.modsrc.id_U2263=1;MCHP.modsrc.id_U2406=1;MCHP.modsrc.id_U2210=1;MCHP.modsrc.id_U2009=1;MCHP.modsrc.id_U2008=1;MCHP.modsrc.id_U2268=1;MCHP.modsrc.id_U2239=1;MCHP.modsrc.id_U2250=1;MCHP.modsrc.id_U2011=2;MCHP.modsrc.id_U2201=8;MCHP.modsrc.id_U2407=1;MCHP.modsrc.id_U2249=8;MCHP.modsrc.id_U2213=5;MCHP.modsrc.id_U2242=1;MCHP.modsrc.id_U2222=1;MCHP.modsrc.id_U2251=1;MCHP.modsrc.id_CoreDebug=1;MCHP.modsrc.id_DWT=1;MCHP.modsrc.id_ETM=1;MCHP.modsrc.id_FPU=1;MCHP.modsrc.id_ITM=1;MCHP.modsrc.id_MPU=1;MCHP.modsrc.id_NVIC=1;MCHP.modsrc.id_SysTick=1;MCHP.modsrc.id_SystemControl=1;MCHP.modsrc.id_TPIU=1;MCHP.modsrc_id.id_U2501.n=1;MCHP.modsrc_id.id_U2501.name='AC';MCHP.modsrc_id.id_U2501.version='1.0.0';MCHP.modsrc_id.id_U2500.n=2;MCHP.modsrc_id.id_U2500.name='ADC';MCHP.modsrc_id.id_U2500.version='1.0.0';MCHP.modsrc_id.id_U2238.n=1;MCHP.modsrc_id.id_U2238.name='AES';MCHP.modsrc_id.id_U2238.version='2.2.0';MCHP.modsrc_id.id_U2003.n=2;MCHP.modsrc_id.id_U2003.name='CAN';MCHP.modsrc_id.id_U2003.version='3.2.1';MCHP.modsrc_id.id_U2225.n=1;MCHP.modsrc_id.id_U2225.name='CCL';MCHP.modsrc_id.id_U2225.version='1.1.0';MCHP.modsrc_id.id_U2015.n=1;MCHP.modsrc_id.id_U2015.name='CMCC';MCHP.modsrc_id.id_U2015.version='6.0.0';MCHP.modsrc_id.id_U2502.n=1;MCHP.modsrc_id.id_U2502.name='DAC';MCHP.modsrc_id.id_U2502.version='1.0.0';MCHP.modsrc_id.id_U2503.n=1;MCHP.modsrc_id.id_U2503.name='DMAC';MCHP.modsrc_id.id_U2503.version='1.0.1';MCHP.modsrc_id.id_U2410.n=1;MCHP.modsrc_id.id_U2410.name='DSU';MCHP.modsrc_id.id_U2410.version='1.0.0';MCHP.modsrc_id.id_U2254.n=1;MCHP.modsrc_id.id_U2254.name='EIC';MCHP.modsrc_id.id_U2254.version='3.0.0';MCHP.modsrc_id.id_U2504.n=1;MCHP.modsrc_id.id_U2504.name='EVSYS';MCHP.modsrc_id.id_U2504.version='1.0.0';MCHP.modsrc_id.id_U2257.n=1;MCHP.modsrc_id.id_U2257.name='FREQM';MCHP.modsrc_id.id_U2257.version='1.1.0';MCHP.modsrc_id.id_U2122.n=1;MCHP.modsrc_id.id_U2122.name='GCLK';MCHP.modsrc_id.id_U2122.version='1.2.0';MCHP.modsrc_id.id_U2005.n=1;MCHP.modsrc_id.id_U2005.name='GMAC';MCHP.modsrc_id.id_U2005.version='1.0.0';MCHP.modsrc_id.id_I7638.n=1;MCHP.modsrc_id.id_I7638.name='HMATRIXB';MCHP.modsrc_id.id_I7638.version='2.1.4';MCHP.modsrc_id.id_U2010.n=1;MCHP.modsrc_id.id_U2010.name='ICM';MCHP.modsrc_id.id_U2010.version='1.2.0';MCHP.modsrc_id.id_U2224.n=1;MCHP.modsrc_id.id_U2224.name='I2S';MCHP.modsrc_id.id_U2224.version='2.0.0';MCHP.modsrc_id.id_U2408.n=1;MCHP.modsrc_id.id_U2408.name='MCLK';MCHP.modsrc_id.id_U2408.version='1.0.0';MCHP.modsrc_id.id_U2409.n=1;MCHP.modsrc_id.id_U2409.name='FUSES';MCHP.modsrc_id.id_U2409.version='1.0.0';MCHP.modsrc_id.id_U2401.n=1;MCHP.modsrc_id.id_U2401.name='OSCCTRL';MCHP.modsrc_id.id_U2401.version='1.0.0';MCHP.modsrc_id.id_U2400.n=1;MCHP.modsrc_id.id_U2400.name='OSC32KCTRL';MCHP.modsrc_id.id_U2400.version='1.0.0';MCHP.modsrc_id.id_U2120.n=1;MCHP.modsrc_id.id_U2120.name='PAC';MCHP.modsrc_id.id_U2120.version='1.2.0';MCHP.modsrc_id.id_U2017.n=1;MCHP.modsrc_id.id_U2017.name='PCC';MCHP.modsrc_id.id_U2017.version='1.1.0';MCHP.modsrc_id.id_U2263.n=1;MCHP.modsrc_id.id_U2263.name='PDEC';MCHP.modsrc_id.id_U2263.version='1.0.0';MCHP.modsrc_id.id_U2406.n=1;MCHP.modsrc_id.id_U2406.name='PM';MCHP.modsrc_id.id_U2406.version='1.0.0';MCHP.modsrc_id.id_U2210.n=1;MCHP.modsrc_id.id_U2210.name='PORT';MCHP.modsrc_id.id_U2210.version='2.2.0';MCHP.modsrc_id.id_U2009.n=1;MCHP.modsrc_id.id_U2009.name='PUKCC';MCHP.modsrc_id.id_U2009.version='2.5.0';MCHP.modsrc_id.id_U2008.n=1;MCHP.modsrc_id.id_U2008.name='QSPI';MCHP.modsrc_id.id_U2008.version='1.6.3';MCHP.modsrc_id.id_U2268.n=1;MCHP.modsrc_id.id_U2268.name='RAMECC';MCHP.modsrc_id.id_U2268.version='1.0.0';MCHP.modsrc_id.id_U2239.n=1;MCHP.modsrc_id.id_U2239.name='RSTC';MCHP.modsrc_id.id_U2239.version='4.0.0';MCHP.modsrc_id.id_U2250.n=1;MCHP.modsrc_id.id_U2250.name='RTC';MCHP.modsrc_id.id_U2250.version='2.1.0';MCHP.modsrc_id.id_U2011.n=2;MCHP.modsrc_id.id_U2011.name='SDHC';MCHP.modsrc_id.id_U2011.version='1.8.3';MCHP.modsrc_id.id_U2201.n=8;MCHP.modsrc_id.id_U2201.name='SERCOM';MCHP.modsrc_id.id_U2201.version='5.0.0';MCHP.modsrc_id.id_U2407.n=1;MCHP.modsrc_id.id_U2407.name='SUPC';MCHP.modsrc_id.id_U2407.version='1.1.0';MCHP.modsrc_id.id_U2249.n=8;MCHP.modsrc_id.id_U2249.name='TC';MCHP.modsrc_id.id_U2249.version='3.0.0';MCHP.modsrc_id.id_U2213.n=5;MCHP.modsrc_id.id_U2213.name='TCC';MCHP.modsrc_id.id_U2213.version='3.1.0';MCHP.modsrc_id.id_U2242.n=1;MCHP.modsrc_id.id_U2242.name='TRNG';MCHP.modsrc_id.id_U2242.version='1.1.0';MCHP.modsrc_id.id_U2222.n=1;MCHP.modsrc_id.id_U2222.name='USB';MCHP.modsrc_id.id_U2222.version='1.2.0';MCHP.modsrc_id.id_U2251.n=1;MCHP.modsrc_id.id_U2251.name='WDT';MCHP.modsrc_id.id_U2251.version='1.1.0';MCHP.modsrc_id.id_CoreDebug.n=1;MCHP.modsrc_id.id_CoreDebug.name='CoreDebug';MCHP.modsrc_id.id_CoreDebug.version='1.0.0';MCHP.modsrc_id.id_DWT.n=1;MCHP.modsrc_id.id_DWT.name='DWT';MCHP.modsrc_id.id_DWT.version='1.0.0';MCHP.modsrc_id.id_ETM.n=1;MCHP.modsrc_id.id_ETM.name='ETM';MCHP.modsrc_id.id_ETM.version='1.0.0';MCHP.modsrc_id.id_FPU.n=1;MCHP.modsrc_id.id_FPU.name='FPU';MCHP.modsrc_id.id_FPU.version='1.0.0';MCHP.modsrc_id.id_ITM.n=1;MCHP.modsrc_id.id_ITM.name='ITM';MCHP.modsrc_id.id_ITM.version='1.0.0';MCHP.modsrc_id.id_MPU.n=1;MCHP.modsrc_id.id_MPU.name='MPU';MCHP.modsrc_id.id_MPU.version='1.0.0';MCHP.modsrc_id.id_NVIC.n=1;MCHP.modsrc_id.id_NVIC.name='NVIC';MCHP.modsrc_id.id_NVIC.version='1.0.0';MCHP.modsrc_id.id_SysTick.n=1;MCHP.modsrc_id.id_SysTick.name='SysTick';MCHP.modsrc_id.id_SysTick.version='1.0.0';MCHP.modsrc_id.id_SystemControl.n=1;MCHP.modsrc_id.id_SystemControl.name='SystemControl';MCHP.modsrc_id.id_SystemControl.version='1.0.0';MCHP.modsrc_id.id_TPIU.n=1;MCHP.modsrc_id.id_TPIU.name='TPIU';MCHP.modsrc_id.id_TPIU.version='1.0.0';MCHP.modsrc_Name.AC.n=1;MCHP.modsrc_Name.AC.id='U2501';MCHP.modsrc_Name.AC.version='1.0.0';MCHP.modsrc_Name.ADC.n=2;MCHP.modsrc_Name.ADC.id='U2500';MCHP.modsrc_Name.ADC.version='1.0.0';MCHP.modsrc_Name.AES.n=1;MCHP.modsrc_Name.AES.id='U2238';MCHP.modsrc_Name.AES.version='2.2.0';MCHP.modsrc_Name.CAN.n=2;MCHP.modsrc_Name.CAN.id='U2003';MCHP.modsrc_Name.CAN.version='3.2.1';MCHP.modsrc_Name.CCL.n=1;MCHP.modsrc_Name.CCL.id='U2225';MCHP.modsrc_Name.CCL.version='1.1.0';MCHP.modsrc_Name.CMCC.n=1;MCHP.modsrc_Name.CMCC.id='U2015';MCHP.modsrc_Name.CMCC.version='6.0.0';MCHP.modsrc_Name.DAC.n=1;MCHP.modsrc_Name.DAC.id='U2502';MCHP.modsrc_Name.DAC.version='1.0.0';MCHP.modsrc_Name.DMAC.n=1;MCHP.modsrc_Name.DMAC.id='U2503';MCHP.modsrc_Name.DMAC.version='1.0.1';MCHP.modsrc_Name.DSU.n=1;MCHP.modsrc_Name.DSU.id='U2410';MCHP.modsrc_Name.DSU.version='1.0.0';MCHP.modsrc_Name.EIC.n=1;MCHP.modsrc_Name.EIC.id='U2254';MCHP.modsrc_Name.EIC.version='3.0.0';MCHP.modsrc_Name.EVSYS.n=1;MCHP.modsrc_Name.EVSYS.id='U2504';MCHP.modsrc_Name.EVSYS.version='1.0.0';MCHP.modsrc_Name.FREQM.n=1;MCHP.modsrc_Name.FREQM.id='U2257';MCHP.modsrc_Name.FREQM.version='1.1.0';MCHP.modsrc_Name.GCLK.n=1;MCHP.modsrc_Name.GCLK.id='U2122';MCHP.modsrc_Name.GCLK.version='1.2.0';MCHP.modsrc_Name.GMAC.n=1;MCHP.modsrc_Name.GMAC.id='U2005';MCHP.modsrc_Name.GMAC.version='1.0.0';MCHP.modsrc_Name.HMATRIXB.n=1;MCHP.modsrc_Name.HMATRIXB.id='I7638';MCHP.modsrc_Name.HMATRIXB.version='2.1.4';MCHP.modsrc_Name.ICM.n=1;MCHP.modsrc_Name.ICM.id='U2010';MCHP.modsrc_Name.ICM.version='1.2.0';MCHP.modsrc_Name.I2S.n=1;MCHP.modsrc_Name.I2S.id='U2224';MCHP.modsrc_Name.I2S.version='2.0.0';MCHP.modsrc_Name.MCLK.n=1;MCHP.modsrc_Name.MCLK.id='U2408';MCHP.modsrc_Name.MCLK.version='1.0.0';MCHP.modsrc_Name.NVMCTRL.n=1;MCHP.modsrc_Name.NVMCTRL.id='U2409';MCHP.modsrc_Name.NVMCTRL.version='1.0.0';MCHP.modsrc_Name.FUSES.n=1;MCHP.modsrc_Name.FUSES.id='U2409';MCHP.modsrc_Name.FUSES.version='1.0.0';MCHP.modsrc_Name.OSCCTRL.n=1;MCHP.modsrc_Name.OSCCTRL.id='U2401';MCHP.modsrc_Name.OSCCTRL.version='1.0.0';MCHP.modsrc_Name.OSC32KCTRL.n=1;MCHP.modsrc_Name.OSC32KCTRL.id='U2400';MCHP.modsrc_Name.OSC32KCTRL.version='1.0.0';MCHP.modsrc_Name.PAC.n=1;MCHP.modsrc_Name.PAC.id='U2120';MCHP.modsrc_Name.PAC.version='1.2.0';MCHP.modsrc_Name.PCC.n=1;MCHP.modsrc_Name.PCC.id='U2017';MCHP.modsrc_Name.PCC.version='1.1.0';MCHP.modsrc_Name.PDEC.n=1;MCHP.modsrc_Name.PDEC.id='U2263';MCHP.modsrc_Name.PDEC.version='1.0.0';MCHP.modsrc_Name.PM.n=1;MCHP.modsrc_Name.PM.id='U2406';MCHP.modsrc_Name.PM.version='1.0.0';MCHP.modsrc_Name.PORT.n=1;MCHP.modsrc_Name.PORT.id='U2210';MCHP.modsrc_Name.PORT.version='2.2.0';MCHP.modsrc_Name.PUKCC.n=1;MCHP.modsrc_Name.PUKCC.id='U2009';MCHP.modsrc_Name.PUKCC.version='2.5.0';MCHP.modsrc_Name.QSPI.n=1;MCHP.modsrc_Name.QSPI.id='U2008';MCHP.modsrc_Name.QSPI.version='1.6.3';MCHP.modsrc_Name.RAMECC.n=1;MCHP.modsrc_Name.RAMECC.id='U2268';MCHP.modsrc_Name.RAMECC.version='1.0.0';MCHP.modsrc_Name.RSTC.n=1;MCHP.modsrc_Name.RSTC.id='U2239';MCHP.modsrc_Name.RSTC.version='4.0.0';MCHP.modsrc_Name.RTC.n=1;MCHP.modsrc_Name.RTC.id='U2250';MCHP.modsrc_Name.RTC.version='2.1.0';MCHP.modsrc_Name.SDHC.n=2;MCHP.modsrc_Name.SDHC.id='U2011';MCHP.modsrc_Name.SDHC.version='1.8.3';MCHP.modsrc_Name.SERCOM.n=8;MCHP.modsrc_Name.SERCOM.id='U2201';MCHP.modsrc_Name.SERCOM.version='5.0.0';MCHP.modsrc_Name.SUPC.n=1;MCHP.modsrc_Name.SUPC.id='U2407';MCHP.modsrc_Name.SUPC.version='1.1.0';MCHP.modsrc_Name.TC.n=8;MCHP.modsrc_Name.TC.id='U2249';MCHP.modsrc_Name.TC.version='3.0.0';MCHP.modsrc_Name.TCC.n=5;MCHP.modsrc_Name.TCC.id='U2213';MCHP.modsrc_Name.TCC.version='3.1.0';MCHP.modsrc_Name.TRNG.n=1;MCHP.modsrc_Name.TRNG.id='U2242';MCHP.modsrc_Name.TRNG.version='1.1.0';MCHP.modsrc_Name.USB.n=1;MCHP.modsrc_Name.USB.id='U2222';MCHP.modsrc_Name.USB.version='1.2.0';MCHP.modsrc_Name.WDT.n=1;MCHP.modsrc_Name.WDT.id='U2251';MCHP.modsrc_Name.WDT.version='1.1.0';MCHP.modsrc_Name.CoreDebug.n=1;MCHP.modsrc_Name.CoreDebug.id='CoreDebug';MCHP.modsrc_Name.CoreDebug.version='1.0.0';MCHP.modsrc_Name.DWT.n=1;MCHP.modsrc_Name.DWT.id='DWT';MCHP.modsrc_Name.DWT.version='1.0.0';MCHP.modsrc_Name.ETM.n=1;MCHP.modsrc_Name.ETM.id='ETM';MCHP.modsrc_Name.ETM.version='1.0.0';MCHP.modsrc_Name.FPU.n=1;MCHP.modsrc_Name.FPU.id='FPU';MCHP.modsrc_Name.FPU.version='1.0.0';MCHP.modsrc_Name.ITM.n=1;MCHP.modsrc_Name.ITM.id='ITM';MCHP.modsrc_Name.ITM.version='1.0.0';MCHP.modsrc_Name.MPU.n=1;MCHP.modsrc_Name.MPU.id='MPU';MCHP.modsrc_Name.MPU.version='1.0.0';MCHP.modsrc_Name.NVIC.n=1;MCHP.modsrc_Name.NVIC.id='NVIC';MCHP.modsrc_Name.NVIC.version='1.0.0';MCHP.modsrc_Name.SysTick.n=1;MCHP.modsrc_Name.SysTick.id='SysTick';MCHP.modsrc_Name.SysTick.version='1.0.0';MCHP.modsrc_Name.SystemControl.n=1;MCHP.modsrc_Name.SystemControl.id='SystemControl';MCHP.modsrc_Name.SystemControl.version='1.0.0';MCHP.modsrc_Name.TPIU.n=1;MCHP.modsrc_Name.TPIU.id='TPIU';MCHP.modsrc_Name.TPIU.version='1.0.0';MCHP.PortBase=32;MCHP.PortPrefixe='P';MCHP.PowerSave=0;MCHP.fcy.GCLKx=reshape([1.2e+08 -1 -1 -1 -1 -1 -1 -1 -1 -1 -1 -1],1,12);MCHP.fcy.MIPS=1.2e+08;MCHP.fcy.APB_HS=1.2e+08;MCHP.fcy.APB_CPU=1.2e+08;MCHP.fcy.AHB_CPU=1.2e+08;MCHP.NTIMERS=8;MCHP.SCCP.nSCCP=0;MCHP.SYS_TICK_TS_Load=9999;MCHP.TimeStepFactor=1;MCHP.INT_PRIORITY_DMA='0';  MCHP_CRC=38223148  BTMODE=Device is in Single Boot (legacy) mode  RES1=Not used  PLLSS=Not used  RES2=Not used  ALTCMPI=Not used  BOREN1=Not used  ALTRB6=Not used  RETCFG=Not used  DFMCY=Not used  BSS2=No Boot Segment  BSEN=No Boot Segment  CWRP=Configuration Segment may be written  CSS=No Protection (other than CWRP)  AIVTDIS=Disabled AIVT  BSLIM=Not used  WDTEN=Disable  BTSWP=BOOTSWP instruction is disabled  DBCC=No Cross Connection between DAC outputs  CTXT1=Not Assigned  CTXT2=Not Assigned  SEQNUM=Not used  nSEQNUM=Not used  BOREN0=Enabled  DMTIVT=Not used  DMTCNT=2^31 (2147483648)  DMTEN=Dead Man Timer is Disabled and can be enabled by software  ON=Not used  USERID=Not used  RESERVED1=Not used  PGL1WAY=Allow only one reconfiguration  FPLLRNG=34-68 MHz Input  FPLLICLK=FRC is input to the System PLL  FPLLMULT=PLL Multiply by 128  UPLLFSEL=USB PLL input is 24 MHz  DMTINTV=Window/Interval value is 127/128 counter value  WDTSPGM=WDT stops during Flash programming  FDMTEN=Deadman Timer is disabled  TRCEN=Trace features in the CPU are enabled  BOOTISA=Boot code and Exception code is MIPS32  FECCCON=ECC and Dynamic ECC are disabled (ECCCON bits are writable)  EXTDDRSIZE=Not used  FSLEEP=Flash is powered down when the device is in Sleep mode  DBGPER=Allow CPU access to all permission regions  EJTAGBEN=Normal EJTAG functionality  TSEQ=Not used  CSEQ=Not used  RWDTPS=1:1048576  RCLKSEL=Always use LPRC  SWDTPS=1:1048576  DMTIVTL=Not used  DMTIVTH=Not used  DMTCNTL=Not used  DMTCNTH=Not used  DMTDIS=Dead Man Timer is Disabled and can be enabled by software  SMBEN=SMBus input threshold is enabled  SPI2PIN=SPI2 uses I/O remap (PPS) pins  CTXT3=Not Assigned  CTXT4=Not Assigned  MBXM0=Mailbox register configured for Master data read (Slave to Master data transfer)  MBXM1=Mailbox register configured for Master data read (Slave to Master data transfer)  MBXM2=Mailbox register configured for Master data read (Slave to Master data transfer)  MBXM3=Mailbox register configured for Master data read (Slave to Master data transfer)  MBXM4=Mailbox register configured for Master data read (Slave to Master data transfer)  MBXM5=Mailbox register configured for Master data read (Slave to Master data transfer)  MBXM6=Mailbox register configured for Master data read (Slave to Master data transfer)  MBXM7=Mailbox register configured for Master data read (Slave to Master data transfer)  MBXM8=Mailbox register configured for Master data read (Slave to Master data transfer)  MBXM9=Mailbox register configured for Master data read (Slave to Master data transfer)  MBXM10=Mailbox register configured for Master data read (Slave to Master data transfer)  MBXM11=Mailbox register configured for Master data read (Slave to Master data transfer)  MBXM12=Mailbox register configured for Master data read (Slave to Master data transfer)  MBXM13=Mailbox register configured for Master data read (Slave to Master data transfer)  MBXM14=Mailbox register configured for Master data read (Slave to Master data transfer)  MBXM15=Mailbox register configured for Master data read (Slave to Master data transfer)  MBXHSA=MSIxMBXD15 assigned to mailbox handshake protocol block A  MBXHSB=MSIxMBXD15 assigned to mailbox handshake protocol block B  MBXHSC=MSIxMBXD15 assigned to mailbox handshake protocol block C  MBXHSD=MSIxMBXD15 assigned to mailbox handshake protocol block D  MBXHSE=MSIxMBXD15 assigned to mailbox handshake protocol block E  MBXHSF=MSIxMBXD15 assigned to mailbox handshake protocol block F  MBXHSG=MSIxMBXD15 assigned to mailbox handshake protocol block G  MBXHSH=MSIxMBXD15 assigned to mailbox handshake protocol block H  HSAEN=Mailbox data flow control handshake protocol block disabled  HSBEN=Mailbox data flow control handshake protocol block disabled  HSCEN=Mailbox data flow control handshake protocol block disabled  HSDEN=Mailbox data flow control handshake protocol block disabled  HSEEN=Mailbox data flow control handshake protocol block disabled  HSFEN=Mailbox data flow control handshake protocol block disabled  HSGEN=Mailbox data flow control handshake protocol block disabled  HSHEN=Mailbox data flow control handshake protocol block disabled  CPRA0=Main core owns pin  CPRA1=Main core owns pin  CPRA2=Main core owns pin  CPRA3=Main core owns pin  CPRA4=Main core owns pin  CPRB0=Main core owns pin  CPRB1=Main core owns pin  CPRB2=Main core owns pin  CPRB3=Main core owns pin  CPRB4=Main core owns pin  CPRB5=Main core owns pin  CPRB6=Main core owns pin  CPRB7=Main core owns pin  CPRB8=Main core owns pin  CPRB9=Main core owns pin  CPRB10=Main core owns pin  CPRB11=Main core owns pin  CPRB12=Main core owns pin  CPRB13=Main core owns pin  CPRB14=Main core owns pin  CPRB15=Main core owns pin  CPRC0=Main core owns pin  CPRC1=Main core owns pin  CPRC2=Main core owns pin  CPRC3=Main core owns pin  CPRC4=Main core owns pin  CPRC5=Main core owns pin  CPRC6=Main core owns pin  CPRC7=Main core owns pin  CPRC8=Main core owns pin  CPRC9=Main core owns pin  CPRC10=Main core owns pin  CPRC11=Main core owns pin  CPRC12=Main core owns pin  CPRC13=Main core owns pin  CPRC14=Main core owns pin  CPRC15=Main core owns pin  CPRD0=Main core owns pin  CPRD1=Main core owns pin  CPRD2=Main core owns pin  CPRD3=Main core owns pin  CPRD4=Main core owns pin  CPRD5=Main core owns pin  CPRD6=Main core owns pin  CPRD7=Main core owns pin  CPRD8=Main core owns pin  CPRD9=Main core owns pin  CPRD10=Main core owns pin  CPRD11=Main core owns pin  CPRD12=Main core owns pin  CPRD13=Main core owns pin  CPRD14=Main core owns pin  CPRD15=Main core owns pin  CPRE0=Main core owns pin  CPRE1=Main core owns pin  CPRE2=Main core owns pin  CPRE3=Main core owns pin  CPRE4=Main core owns pin  CPRE5=Main core owns pin  CPRE6=Main core owns pin  CPRE7=Main core owns pin  CPRE8=Main core owns pin  CPRE9=Main core owns pin  CPRE10=Main core owns pin  CPRE11=Main core owns pin  CPRE12=Main core owns pin  CPRE13=Main core owns pin  CPRE14=Main core owns pin  CPRE15=Main core owns pin  S1FNOSC=Internal Fast RC (FRC) Oscillator with postscaler  S1IESO=Start up with FRC; then switch  S1OSCIOFNC=OSC2 is clock output  S1FCKSM=Both Clock switching and Fail-safe Clock Monitor are disabled  S1PLLKEN=S1PLLKEN_ON  S1RWDTPS=1:1048576  S1RCLKSEL=Always use LPRC  S1WINDIS=Watchdog Timer operates in Non-Window mode  S1WDTWIN=WDT Window is 25% of WDT period  S1SWDTPS=1:1048576  S1FWDTEN=use WDTCON.ON bit  S1ICS=Communicate on PGC1 and PGD1  S1DEBUG=Not used  S1ISOLAT=The Secondary can operate (in debug mode) even if the SLVEN bit in the MSI is zero  S1NOBTSWP=BOOTSWP instruction is disabled  S1ALTI2C1=I2C1 mapped to SDA1/SCL1 pins  S1SPI1PIN=Secondary SPI1 uses I/O remap (PPS) pins  S1SSRE=Slave generated resets will reset the Slave Enable Bit in the MSI module  S1MSRE=The Main software oriented RESET events (RESET Op-Code; Watchdog timeout; TRAP reset; illegalInstruction) will also cause the Secondary subsystem to reset  S1CTXT1=Not Assigned  S1CTXT2=Not Assigned  S1CTXT3=Not Assigned  S1CTXT4=Not Assigned  BORLVL=BOR trip point is 2.96 V  BSSO=Normal startup operation after reset; execute instruction at 0x000000  MCA=Flash read accesses are 2 cycle to support maximum processor frequency of operation  MAXTEMP=20 ns flash access  CFGAN14=Device pin is input to AN14  CFGAN15=Device pin is input to AN15  S1IOL1WAY=Allow only one reconfiguration  S1BSSO=Normal startup operation after reset; execute instruction at 0x000000  S1BACKBUG=Not used  BISTDIS=mBIST on reset feature disabled  NOBTSWP=BOOTSWP instruction is disabled  S1BISTDIS=Secondary BIST on reset feature disabled  S1DMTIVTL=Not used  S1DMTIVTH=Not used  S1DMTCNTL=Not used  S1DMTCNTH=Not used  S1DMTDIS=Secondary Dead Man Timer is Disabled and can be enabled by software  BSEQ=Not used  IBSEQ=Not used  SMB3EN=SMBus 3.0 input levels  FUSBIDIO2=USBID pin is controlled by the USB2 module  FVBUSIO2=VBUSON pin is controlled by the USB2 module  FUSBIDIO1=USBID pin is controlled by the USB1 module  FVBUSIO1=VBUSON pin is controlled by the USB1 module  VBATBOREN=Enable ZPBOR during VBAT Mode  FDSEN=Enable DSEN bit in DSCON  BORSEL=BOR trip voltage 2.1v (Non-OPAMP deviced operation)  POSCFGAIN=Gain is G3  POSCAGCDLY=Settling time = 25ms x AGCRNG  POSCAGCRNG=Range 1x  POSCAGC=Automatic Gain Control for Oscillator  FDBGWP=Not used
      settings: SourceProductName=MPLAB Device Blocks for Simulink
  Port Info : MCHP_Blockset/System Info/Port Info  MCHP_MASTERLINK=mcb_microchip_pmsm_foc_sensorless_SAME54_pot1/Configurations/Microchip Master
      settings: SourceProductName=MPLAB Device Blocks for Simulink
  UART Configuration1 : MCHP_Blockset/BUS UART/UART Configuration  UART_REF=SERCOM USART 2  BAUD_Choice=Dynamic Options  BAUD_Choice_TXT="1200000         [-0.00%]"  BAUD_Choice_IR=Dynamic Options  BAUD_Choice_IR_TXT=[]  BAUD_Custom=1000000  INT_PRIORITY=3  ALT_IO=on  PIN_RX=Dynamic Options  PIN_RX_TXT=PA13 / Pin[61] / pad1  PIN_TX=Dynamic Options  PIN_TX_TXT=PA12 / Pin[60] / pad0  MCHP_PORT={UART2 Rx}{SERCOM2_PAD1}3:0:P13;{UART2 Tx}{SERCOM2_PAD0}3:1:P12;  MCHP_MASTERLINK=mcb_microchip_pmsm_foc_sensorless_SAME54_pot/Configurations/Microchip Master  MCHP_COM_ExtPil=off  TX_IMPLEMENTATION=Circular Buffer  TX_IMPLEMENTATION_default=Circular Buffer  TX_INT_PRIORITY=4  TX_INT_WHEN=is empty  TX_INT_WHEN_default=is empty & last char is sent  TX_CIRCULAR_SIZE=512  TX_DMA_CHANNEL=0  TX_DMA_SIZE=[]  TX_TASK_PROTECTION=Delay tasks (default)  TX_INTERRUPT_PROTECTION=Do not send on conflict (default)  TX_INTERRUPT_PROTECTION_default=Do not send on conflict (default)  RX_IMPLEMENTATION=Circular Buffer  RX_IMPLEMENTATION_default=Circular Buffer  RX_INT_PRIORITY=4  RX_INT_WHEN=receive 1 character  RX_CIRCULAR_SIZE=512  RX_DMA_CHANNEL=0  RX_DMA_SIZE=0  DuplexMode=Full duplex (default)  PIN_RX_Inv=off  PIN_TX_Inv=off  PIN_RXTX_Inv=off  ParityBit=No parity (default)  StopBit=1 stop bit (default)  IRDA=off  IdleTime_choice=Dynamic Options  IdleTime_choice_TXT=0  IdleTime_custom=2/50  FlowControl=None  PIN_CTS=Dynamic Options  PIN_CTS_TXT=PA10 / Pin[35] / pad2  PIN_RTS=Dynamic Options  PIN_RTS_TXT=PA11 / Pin[36] / pad3  PIN_DSR=Dynamic Options  PIN_DSR_TXT=Dynamic Options  PIN_DTR=Dynamic Options  PIN_DTR_TXT=Dynamic Options  InitSequence_chkbox=off  BAUD_Choice_InitSeq=Dynamic Options  BAUD_Choice_InitSeq_TXT="115200         [+0.03%]"  BAUD_Choice_IR_InitSeq=Dynamic Options  BAUD_Choice_IR_InitSeq_TXT=0  BAUD_Custom_InitSeq=0  InitSequence='Hello World'
      settings: SourceProductName=MPLAB Device Blocks for Simulink
